simulink model "TLC_Network"  (R2022b)
settings: Solver=VariableStepAuto  StartTime=0.0  StopTime=2  RelTol=1e-3
(part 1 of 2)
settings Model: Creator=Stefano  LastModifiedBy=stefanopanzieri
settings SolverCC: AlgebraicLoopSolver=TrustRegion
settings DebuggingCC: UnconnectedInputMsg=warning  UnconnectedOutputMsg=warning  UnconnectedLineMsg=warning  SFMachineParentedDataDiag=warning
settings ModelReferenceCC: EnableRefExpFcnMdlSchedulingChecks=on
settings SFSimCC: CustomCodeUndefinedFunction=UseInterfaceOnly
settings RTWCC: DLArmComputeVersion=19.05

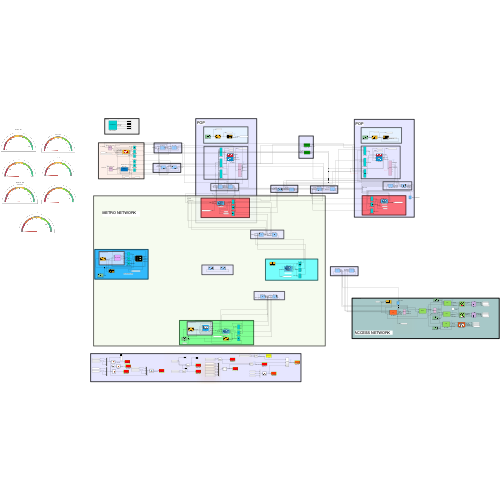
[thumbnail: Simulink's stored preview of the top-level diagram]
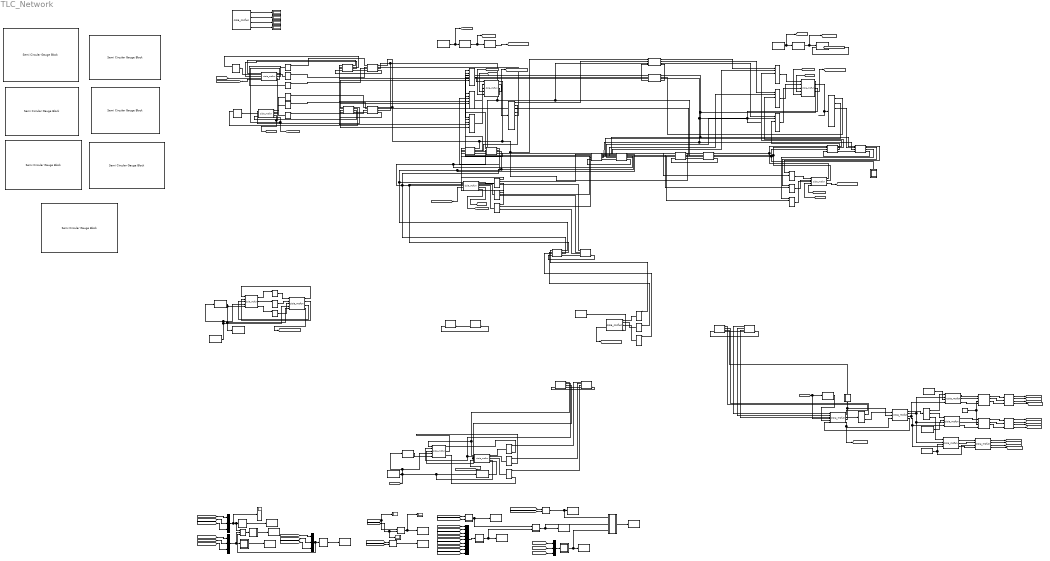
== system TLC_Network ==
  note: POP
  note: ACCESS NETWORK
  note: METRO NETWORK
  note: Web App Firewalls
  note: Core Router/Provider Edge
  note: Distribution Router
  note: Access Router
  note: Border Router
  note: Firewall, IPS/IDS, Malware Detection&Protection
  note: Border Router
  note: Core Network Room
  note: Core Network Room
  note: ACCESS NETWORK
  note: POP
  note: MASTER
  5G_CU_DU_Server_1 (160) : M-S-Function  FunctionName=cisia_msfun  Parameters=Parameter1, Parameter2, Parameter3, resources, Parameter10, codeupdate, step_received, step_computed, dynamic_computed, step_sended, id_entity, id_project, id_type, name_type, color  mask(S-function:msfcn_unit_delay){Parameter1='5G_CU_DU_Server_1', Parameter2=1, Parameter3='ORO', resources=, Parameter10=off, codeupdate=off, step_received=|, step_computed=, dynamic_computed=, step_sended=|, id_entity=160, id_project=6, id_type=40, name_type=App_Server, color=#00AAFF}
      mask step_received=|
      | Connection=max(Connection_init,TLC_CONN);
      | TLC_services=max(TLC_services_init,TLC_SERVICE);
      | TLC_services=mod(TLC_services,10);
      | TLC_revoke=floor(TLC_SERVICE/10);
      |
      | Mechanical_Fault=max([Mechanical_Fault Mechanical_Fault_init]);
      |
      | %if strcmp(name_entity,"BlockChainServer") && (cisia.major_time>=2)
      |  % Dos_attack=1;
      |  %TLC_revoke(9)=1;
      |  %TLC_services(9)=0;
      | %end
      |
      |
      | Cyber_Fault=max(CYBER_FAULT, transpose([Dos_attack   MITM_attack Virus_Attack Port_Scan_Attack  BGP_hijacking BotNet_Attack Data_Corruption SW_Change Config_Change Port_Saturation]));
      |
      | Service_Fault=max(abs(Consumed_Services.*TLC_services-Consumed_Services));
      | Redundancy_Fault=max(abs(Consumed_Services.*TLC_CONN-Consumed_Services));
      |
      | Conn_Fault=max([Dos_attack  Mechanical_Fault  1-POWER 1-ROOM_QoS] );
      |
      |
      | Operative_Level=(1-Conn_Fault)*(1-0.5*max(Cyber_Fault))*(1-Service_Fault)*max(max(TLC_CONN),0.5);
      mask step_sended=|
      | TLC_CONN=Connection*(1-Conn_Fault);
      | TLC_SERVICE=TLC_services*(1-Conn_Fault)*(1-Service_Fault)*(1-syslog_adm_login)+10*TLC_revoke;
      | CYBER_FAULT=Cyber_Fault*(1-Conn_Fault);
      mask prompts: Parameter1 "entity name"; Parameter2 "sampling time"; Parameter3 "project"; resources "input resources and state variables"; Parameter10 "Bring state variables to output"; codeupdate "update code from mask"
      mask help: This is a level-2 MATLAB file S-function which demonstrates CISIA entity
      mask DialogControl Container1 Prompt: All parameters
      mask Display: image('Icons/App_Server.png')
  5G_Core_1 (198) : M-S-Function  FunctionName=cisia_msfun  Parameters=Parameter1, Parameter2, Parameter3, resources, Parameter10, codeupdate, step_received, step_computed, dynamic_computed, step_sended, id_entity, id_project, id_type, name_type, color  mask(S-function:msfcn_unit_delay){Parameter1='5G_Core_1', Parameter2=1, Parameter3='ORO', resources=, Parameter10=off, codeupdate=off, step_received=|, step_computed=, dynamic_computed=, step_sended=|, id_entity=198, id_project=6, id_type=38, name_type=5G_Core, color=#E7A6FF}
      mask step_received=|
      | Connection=max(Connection_init,TLC_CONN);
      | TLC_services=max(TLC_services_init,TLC_SERVICE);
      | TLC_services=mod(TLC_services,10);
      | TLC_revoke=floor(TLC_SERVICE/10);
      | Mechanical_Fault=max([Mechanical_Fault Mechanical_Fault_init]);
      |
      | Cyber_Fault=max(CYBER_FAULT, transpose([Dos_attack   MITM_attack Virus_Attack Port_Scan_Attack  BGP_hijacking BotNet_Attack Data_Corruption SW_Change Config_Change Port_Saturation]));
      |
      |
      |
      | %if (cisia.major_time)>=2
      |    %Dos_attack=1;
      |    %TLC_services(5)=0;
      |   %TLC_revoke(5)=1;
      | %end
      |
      |
      | Conn_Fault=max([Dos_attack  Mechanical_Fault  1-POWER 1-ROOM_QoS] );
      |
      | Service_Fault=max(abs(Consumed_Services.*TLC_services-Consumed_Services));
      | Redundancy_Fault=max(abs(Consumed_Services.*TLC_CONN-Consumed_Services));
      |
      | Operative_Level=(1-Conn_Fault)*(1-0.5*max(Cyber_Fault))*(1-Service_Fault);
      mask step_sended=|
      | TLC_CONN=Connection*(1-Conn_Fault);
      | TLC_SERVICE=TLC_services*(1-Conn_Fault)*(1-Service_Fault)*(1 -syslog_adm_login)+10*TLC_revoke;
      | %TLC_SERVICE=TLC_services
      | CYBER_FAULT=Cyber_Fault*(1-Conn_Fault);
      mask prompts: Parameter1 "entity name"; Parameter2 "sampling time"; Parameter3 "project"; resources "input resources and state variables"; Parameter10 "Bring state variables to output"; codeupdate "update code from mask"
      mask help: This is a level-2 MATLAB file S-function which demonstrates CISIA entity
      mask DialogControl Container1 Prompt: All parameters
      mask Display: disp('RFI_Sist_Informativo_1')
  ANTENNA_1 (56) : M-S-Function  FunctionName=cisia_msfun  Parameters=Parameter1, Parameter2, Parameter3, resources, Parameter10, codeupdate, step_received, step_computed, dynamic_computed, step_sended, id_entity, id_project, id_type, name_type, color  mask(S-function:msfcn_unit_delay){Parameter1='ANTENNA_1', Parameter2=1, Parameter3='ORO', resources=, Parameter10=off, codeupdate=off, step_received=|, step_computed=, dynamic_computed=, step_sended=|, id_entity=56, id_project=6, id_type=13, name_type=RU-DU_ANTENNA, color=#90DB5A}
      mask step_received=|
      | Connection=max(Connection_init,NGPON_CONN);
      | TLC_services=max(TLC_services_init,TLC_SERVICE);
      | TLC_services=mod(TLC_services,10);
      | TLC_revoke=floor(TLC_SERVICE/10);
      |
      | Cyber_Fault=max(CYBER_FAULT, transpose([Dos_attack   MITM_attack Virus_Attack Port_Scan_Attack  BGP_hijacking BotNet_Attack Data_Corruption SW_Change Config_Change Port_Saturation]));
      |
      | % Vale 1 in presenza di fault
      | Conn_Fault=max([Dos_attack  Mechanical_Fault  1-POWER] );
      |
      | Service_Fault=max(abs(Consumed_Services.*TLC_services-Consumed_Services));
      | Redundancy_Fault=max(abs(Consumed_Services.*NGPON_CONN-Consumed_Services));
      |
      |
      | Operative_Level=(1-Conn_Fault)*max(max(NGPON_CONN),0.5)*((2*(1-Service_Fault)+(1-Redundancy_Fault))/3);
      |
      | % Il servizio utilizzato
      | My_Service=max([(1-Service_Fault) (1-Redundancy_Fault)/2]);
      mask step_sended=|
      | R_CONN=Connection*(1-Conn_Fault);
      | TLC_SERVICE=TLC_services*(1-Conn_Fault)+10*TLC_revoke;
      |
      | Cyber_Transmitted=min(Cyber_Fault, transpose([0 0 1 0 1 1 0 0 0 1]));
      | CYBER_FAULT=Cyber_Transmitted*(1-Conn_Fault);
      |
      |
      | RF_QoS=My_Service;
      mask prompts: Parameter1 "entity name"; Parameter2 "sampling time"; Parameter3 "project"; resources "input resources and state variables"; Parameter10 "Bring state variables to output"; codeupdate "update code from mask"
      mask help: This is a level-2 MATLAB file S-function which demonstrates CISIA entity
      mask DialogControl Container1 Prompt: All parameters
      mask Display: image('Icons/RU-DU_ANTENNA.png')
  ANTENNA_2 (60) : M-S-Function  FunctionName=cisia_msfun  Parameters=Parameter1, Parameter2, Parameter3, resources, Parameter10, codeupdate, step_received, step_computed, dynamic_computed, step_sended, id_entity, id_project, id_type, name_type, color  mask(S-function:msfcn_unit_delay){Parameter1='ANTENNA_2', Parameter2=1, Parameter3='ORO', resources=, Parameter10=off, codeupdate=off, step_received=|, step_computed=, dynamic_computed=, step_sended=|, id_entity=60, id_project=6, id_type=13, name_type=RU-DU_ANTENNA, color=#90DB5A}
      mask step_received=|
      | Connection=max(Connection_init,NGPON_CONN);
      | TLC_services=max(TLC_services_init,TLC_SERVICE);
      | TLC_services=mod(TLC_services,10);
      | TLC_revoke=floor(TLC_SERVICE/10);
      |
      | Cyber_Fault=max(CYBER_FAULT, transpose([Dos_attack   MITM_attack Virus_Attack Port_Scan_Attack  BGP_hijacking BotNet_Attack Data_Corruption SW_Change Config_Change Port_Saturation]));
      |
      | % Vale 1 in presenza di fault
      | Conn_Fault=max([Dos_attack  Mechanical_Fault  1-POWER] );
      |
      | Service_Fault=max(abs(Consumed_Services.*TLC_services-Consumed_Services));
      | Redundancy_Fault=max(abs(Consumed_Services.*NGPON_CONN-Consumed_Services));
      |
      |
      | Operative_Level=(1-Conn_Fault)*max(max(NGPON_CONN),0.5)*((2*(1-Service_Fault)+(1-Redundancy_Fault))/3);
      |
      | % Il servizio utilizzato
      | My_Service=max([(1-Service_Fault) (1-Redundancy_Fault)/2]);
      mask step_sended=|
      | R_CONN=Connection*(1-Conn_Fault);
      | TLC_SERVICE=TLC_services*(1-Conn_Fault)+10*TLC_revoke;
      |
      | Cyber_Transmitted=min(Cyber_Fault, transpose([0 0 1 0 1 1 0 0 0 1]));
      | CYBER_FAULT=Cyber_Transmitted*(1-Conn_Fault);
      |
      |
      | RF_QoS=My_Service;
      mask prompts: Parameter1 "entity name"; Parameter2 "sampling time"; Parameter3 "project"; resources "input resources and state variables"; Parameter10 "Bring state variables to output"; codeupdate "update code from mask"
      mask help: This is a level-2 MATLAB file S-function which demonstrates CISIA entity
      mask DialogControl Container1 Prompt: All parameters
      mask Display: image('Icons/RU-DU_ANTENNA.png')
  ASR9006_1 (9) : M-S-Function  FunctionName=cisia_msfun  Parameters=Parameter1, Parameter2, Parameter3, resources, Parameter10, codeupdate, step_received, step_computed, dynamic_computed, step_sended, id_entity, id_project, id_type, name_type, color  mask(S-function:msfcn_unit_delay){Parameter1='ASR9006_1', Parameter2=1, Parameter3='ORO', resources=, Parameter10=off, codeupdate=off, step_received=|, step_computed=, dynamic_computed=, step_sended=|, id_entity=9, id_project=6, id_type=3, name_type=CISCO_router, color=#4DBEEE}
      mask step_received=|
      | Connection=max(Connection_init,TLC_CONN);
      | TLC_services=max(TLC_services_init,TLC_SERVICE);
      | TLC_services=mod(TLC_services,10);
      | TLC_revoke=floor(TLC_SERVICE/10);
      |
      | Cyber_Fault=max(CYBER_FAULT, transpose([Dos_attack   MITM_attack Virus_Attack Port_Scan_Attack  BGP_hijacking BotNet_Attack Data_Corruption SW_Change Config_Change Port_Saturation]));
      |
      |
      | Conn_Fault=max([Dos_attack BGP_hijacking Route_Poisoning Interface_Down Mechanical_Fault  1-POWER 1-ROOM_QoS Earthquake_Fault] );
      |
      | Room_Fault=1-ROOM_QoS;
      |
      | Operative_Level=(1-Room_Fault)*(1-Conn_Fault)*max(max(TLC_services),0.5)*(1-0.5*max(Cyber_Fault));
      mask step_sended=|
      | TLC_CONN=Connection*(1-Conn_Fault);
      | TLC_SERVICE=TLC_services*(1-Room_Fault)*(1-Conn_Fault)*(1-syslog_adm_login)+10*TLC_revoke;
      |
      |
      | Cyber_Transmitted=min(Cyber_Fault, transpose([0 0 1 0 1 1 0 0 0 1]));
      |
      | CYBER_FAULT=Cyber_Transmitted*(1-Conn_Fault);
      |
      | ROUTING_QoS=Operative_Level;
      mask prompts: Parameter1 "entity name"; Parameter2 "sampling time"; Parameter3 "project"; resources "input resources and state variables"; Parameter10 "Bring state variables to output"; codeupdate "update code from mask"
      mask help: This is a level-2 MATLAB file S-function which demonstrates CISIA entity
      mask DialogControl Container1 Prompt: All parameters
      mask Display: image('Icons/CISCO_router.png')
  ASR9006_2 (10) : M-S-Function  FunctionName=cisia_msfun  Parameters=Parameter1, Parameter2, Parameter3, resources, Parameter10, codeupdate, step_received, step_computed, dynamic_computed, step_sended, id_entity, id_project, id_type, name_type, color  mask(S-function:msfcn_unit_delay){Parameter1='ASR9006_2', Parameter2=1, Parameter3='ORO', resources=, Parameter10=off, codeupdate=off, step_received=|, step_computed=, dynamic_computed=, step_sended=|, id_entity=10, id_project=6, id_type=3, name_type=CISCO_router, color=#4DBEEE}
      mask step_received=|
      | Connection=max(Connection_init,TLC_CONN);
      | TLC_services=max(TLC_services_init,TLC_SERVICE);
      | TLC_services=mod(TLC_services,10);
      | TLC_revoke=floor(TLC_SERVICE/10);
      |
      | Cyber_Fault=max(CYBER_FAULT, transpose([Dos_attack   MITM_attack Virus_Attack Port_Scan_Attack  BGP_hijacking BotNet_Attack Data_Corruption SW_Change Config_Change Port_Saturation]));
      |
      |
      | Conn_Fault=max([Dos_attack BGP_hijacking Route_Poisoning Interface_Down Mechanical_Fault  1-POWER 1-ROOM_QoS Earthquake_Fault] );
      |
      | Room_Fault=1-ROOM_QoS;
      |
      | Operative_Level=(1-Room_Fault)*(1-Conn_Fault)*max(max(TLC_services),0.5)*(1-0.5*max(Cyber_Fault));
      mask step_sended=|
      | TLC_CONN=Connection*(1-Conn_Fault);
      | TLC_SERVICE=TLC_services*(1-Room_Fault)*(1-Conn_Fault)*(1-syslog_adm_login)+10*TLC_revoke;
      |
      |
      | Cyber_Transmitted=min(Cyber_Fault, transpose([0 0 1 0 1 1 0 0 0 1]));
      |
      | CYBER_FAULT=Cyber_Transmitted*(1-Conn_Fault);
      |
      | ROUTING_QoS=Operative_Level;
      mask prompts: Parameter1 "entity name"; Parameter2 "sampling time"; Parameter3 "project"; resources "input resources and state variables"; Parameter10 "Bring state variables to output"; codeupdate "update code from mask"
      mask help: This is a level-2 MATLAB file S-function which demonstrates CISIA entity
      mask DialogControl Container1 Prompt: All parameters
      mask Display: image('Icons/CISCO_router.png')
  ASR903_1 (5) : M-S-Function  FunctionName=cisia_msfun  Parameters=Parameter1, Parameter2, Parameter3, resources, Parameter10, codeupdate, step_received, step_computed, dynamic_computed, step_sended, id_entity, id_project, id_type, name_type, color  mask(S-function:msfcn_unit_delay){Parameter1='ASR903_1', Parameter2=1, Parameter3='ORO', resources=, Parameter10=off, codeupdate=off, step_received=|, step_computed=, dynamic_computed=, step_sended=|, id_entity=5, id_project=6, id_type=3, name_type=CISCO_router, color=#4DBEEE}
      mask step_received=|
      | Connection=max(Connection_init,TLC_CONN);
      | TLC_services=max(TLC_services_init,TLC_SERVICE);
      | TLC_services=mod(TLC_services,10);
      | TLC_revoke=floor(TLC_SERVICE/10);
      |
      | Cyber_Fault=max(CYBER_FAULT, transpose([Dos_attack   MITM_attack Virus_Attack Port_Scan_Attack  BGP_hijacking BotNet_Attack Data_Corruption SW_Change Config_Change Port_Saturation]));
      |
      |
      | Conn_Fault=max([Dos_attack BGP_hijacking Route_Poisoning Interface_Down Mechanical_Fault  1-POWER 1-ROOM_QoS Earthquake_Fault] );
      |
      | Room_Fault=1-ROOM_QoS;
      |
      | Operative_Level=(1-Room_Fault)*(1-Conn_Fault)*max(max(TLC_services),0.5)*(1-0.5*max(Cyber_Fault));
      mask step_sended=|
      | TLC_CONN=Connection*(1-Conn_Fault);
      | TLC_SERVICE=TLC_services*(1-Room_Fault)*(1-Conn_Fault)*(1-syslog_adm_login)+10*TLC_revoke;
      |
      |
      | Cyber_Transmitted=min(Cyber_Fault, transpose([0 0 1 0 1 1 0 0 0 1]));
      |
      | CYBER_FAULT=Cyber_Transmitted*(1-Conn_Fault);
      |
      | ROUTING_QoS=Operative_Level;
      mask prompts: Parameter1 "entity name"; Parameter2 "sampling time"; Parameter3 "project"; resources "input resources and state variables"; Parameter10 "Bring state variables to output"; codeupdate "update code from mask"
      mask help: This is a level-2 MATLAB file S-function which demonstrates CISIA entity
      mask DialogControl Container1 Prompt: All parameters
      mask Display: image('Icons/CISCO_router.png')
  ASR920_1 (7) : M-S-Function  FunctionName=cisia_msfun  Parameters=Parameter1, Parameter2, Parameter3, resources, Parameter10, codeupdate, step_received, step_computed, dynamic_computed, step_sended, id_entity, id_project, id_type, name_type, color  mask(S-function:msfcn_unit_delay){Parameter1='ASR920_1', Parameter2=1, Parameter3='ORO', resources=, Parameter10=off, codeupdate=off, step_received=|, step_computed=, dynamic_computed=, step_sended=|, id_entity=7, id_project=6, id_type=3, name_type=CISCO_router, color=#4DBEEE}
      mask step_received=|
      | Connection=max(Connection_init,TLC_CONN);
      | TLC_services=max(TLC_services_init,TLC_SERVICE);
      | TLC_services=mod(TLC_services,10);
      | TLC_revoke=floor(TLC_SERVICE/10);
      |
      | Cyber_Fault=max(CYBER_FAULT, transpose([Dos_attack   MITM_attack Virus_Attack Port_Scan_Attack  BGP_hijacking BotNet_Attack Data_Corruption SW_Change Config_Change Port_Saturation]));
      |
      |
      | Conn_Fault=max([Dos_attack BGP_hijacking Route_Poisoning Interface_Down Mechanical_Fault  1-POWER 1-ROOM_QoS Earthquake_Fault] );
      |
      | Room_Fault=1-ROOM_QoS;
      |
      | Operative_Level=(1-Room_Fault)*(1-Conn_Fault)*max(max(TLC_services),0.5)*(1-0.5*max(Cyber_Fault));
      mask step_sended=|
      | TLC_CONN=Connection*(1-Conn_Fault);
      | TLC_SERVICE=TLC_services*(1-Room_Fault)*(1-Conn_Fault)*(1-syslog_adm_login)+10*TLC_revoke;
      |
      |
      | Cyber_Transmitted=min(Cyber_Fault, transpose([0 0 1 0 1 1 0 0 0 1]));
      |
      | CYBER_FAULT=Cyber_Transmitted*(1-Conn_Fault);
      |
      | ROUTING_QoS=Operative_Level;
      mask prompts: Parameter1 "entity name"; Parameter2 "sampling time"; Parameter3 "project"; resources "input resources and state variables"; Parameter10 "Bring state variables to output"; codeupdate "update code from mask"
      mask help: This is a level-2 MATLAB file S-function which demonstrates CISIA entity
      mask DialogControl Container1 Prompt: All parameters
      mask Display: image('Icons/CISCO_router.png')
  Alcatel_1 (26) : M-S-Function  FunctionName=cisia_msfun  Parameters=Parameter1, Parameter2, Parameter3, resources, Parameter10, codeupdate, step_received, step_computed, dynamic_computed, step_sended, id_entity, id_project, id_type, name_type, color  mask(S-function:msfcn_unit_delay){Parameter1='Alcatel_1', Parameter2=1, Parameter3='ORO', resources=, Parameter10=off, codeupdate=off, step_received=|, step_computed=, dynamic_computed=, step_sended=|, id_entity=26, id_project=6, id_type=5, name_type=Alcatel7750, color=#ACBD7E}
      mask step_received=|
      | Connection=max(Connection_init,TLC_CONN);
      | TLC_services=max(TLC_services_init,TLC_SERVICE);
      | TLC_services=mod(TLC_services,10);
      | TLC_revoke=floor(TLC_SERVICE/10);
      |
      | Cyber_Fault=max(CYBER_FAULT, transpose([Dos_attack   MITM_attack Virus_Attack Port_Scan_Attack  BGP_hijacking BotNet_Attack Data_Corruption SW_Change Config_Change Port_Saturation]));
      |
      | Conn_Fault=max([Dos_attack  Mechanical_Fault  1-POWER 1-ROOM_QoS] );
      |
      |
      | Operative_Level=(1-Conn_Fault)*(1-0.5*max(Cyber_Fault))*max(max(TLC_services),0.5);
      mask step_sended=|
      | TLC_CONN=Connection*(1-Conn_Fault);
      | TLC_SERVICE=TLC_services*(1-Conn_Fault)+TLC_revoke*10;
      | CYBER_FAULT=Cyber_Fault*(1-Conn_Fault);
      |
      | ROUTING_QoS=Operative_Level;
      mask prompts: Parameter1 "entity name"; Parameter2 "sampling time"; Parameter3 "project"; resources "input resources and state variables"; Parameter10 "Bring state variables to output"; codeupdate "update code from mask"
      mask help: This is a level-2 MATLAB file S-function which demonstrates CISIA entity
      mask DialogControl Container1 Prompt: All parameters
      mask Display: image('Icons/Alcatel7750.png')
  BIGP_2 (35) : M-S-Function  FunctionName=cisia_msfun  Parameters=Parameter1, Parameter2, Parameter3, resources, Parameter10, codeupdate, step_received, step_computed, dynamic_computed, step_sended, id_entity, id_project, id_type, name_type, color  mask(S-function:msfcn_unit_delay){Parameter1='BIGP_2', Parameter2=1, Parameter3='ORO', resources=, Parameter10=off, codeupdate=off, step_received=|, step_computed=, dynamic_computed=, step_sended=|, id_entity=35, id_project=6, id_type=7, name_type=F5BIGP, color=#0072BD}
      mask step_received=|
      | Connection=max(Connection_init,TLC_CONN);
      | TLC_services=max(TLC_services_init,TLC_SERVICE);
      | TLC_services=mod(TLC_services,10);
      | TLC_revoke=floor(TLC_SERVICE/10);
      |
      | Cyber_Fault=max(CYBER_FAULT, transpose([Dos_attack   MITM_attack Virus_Attack Port_Scan_Attack  BGP_hijacking BotNet_Attack Data_Corruption SW_Change Config_Change Port_Saturation]));
      |
      | Conn_Fault=max([Dos_attack  Mechanical_Fault  1-POWER 1-ROOM_QoS] );
      |
      | Service_Fault=max(abs(Consumed_Services.*TLC_services-Consumed_Services));
      | Redundancy_Fault=max(abs(Consumed_Services.*TLC_CONN-Consumed_Services));
      |
      | %Operative_Level=(1-Conn_Fault)*((2*(1-Service_Fault)+(1-Redundancy_Fault))/3);
      | Operative_Level=(1-Conn_Fault)*(1-0.5*max(Cyber_Fault))*(1-Service_Fault)*max(max(TLC_CONN),0.5);
      mask step_sended=|
      | TLC_CONN=Connection*(1-Conn_Fault);
      | TLC_SERVICE=TLC_services*(1-Conn_Fault)*(1-Service_Fault)+10*TLC_revoke;
      |
      | Cyber_Transmitted=min(Cyber_Fault, transpose([0 0 1 0 1 1 0 0 0 1]));
      |
      | CYBER_FAULT=Cyber_Transmitted*(1-Conn_Fault);
      mask prompts: Parameter1 "entity name"; Parameter2 "sampling time"; Parameter3 "project"; resources "input resources and state variables"; Parameter10 "Bring state variables to output"; codeupdate "update code from mask"
      mask help: This is a level-2 MATLAB file S-function which demonstrates CISIA entity
      mask DialogControl Container1 Prompt: All parameters
      mask Display: disp('F5BIGP')
  BLM_1500 (91) : M-S-Function  FunctionName=cisia_msfun  Parameters=Parameter1, Parameter2, Parameter3, resources, Parameter10, codeupdate, step_received, step_computed, dynamic_computed, step_sended, id_entity, id_project, id_type, name_type, color  mask(S-function:msfcn_unit_delay){Parameter1='BLM_1500', Parameter2=1, Parameter3='ORO', resources=, Parameter10=off, codeupdate=off, step_received=|, step_computed=, dynamic_computed=, step_sended=|, id_entity=91, id_project=6, id_type=4, name_type=OLT, color=#FF6929}
      mask step_received=|
      | Connection=max(Connection_init,TLC_CONN);
      | TLC_services=max(TLC_services_init,TLC_SERVICE);
      | TLC_services=mod(TLC_services,10);
      | TLC_revoke=floor(TLC_SERVICE/10);
      |
      | Cyber_Fault=max(CYBER_FAULT, transpose([Dos_attack   MITM_attack Virus_Attack Port_Scan_Attack  BGP_hijacking BotNet_Attack Data_Corruption SW_Change Config_Change Port_Saturation]));
      |
      |
      | % Vale 1 in presenza di fault
      | Conn_Fault=max([Dos_attack  Mechanical_Fault  1-POWER 1-ROOM_QoS] );
      |
      |
      | Service_Fault=max(abs(Consumed_Services.*TLC_services-Consumed_Services));
      |
      |
      | Redundancy_Fault=max(abs(Consumed_Services.*TLC_CONN-Consumed_Services));
      |
      | Operative_Level=(1-Conn_Fault)*(1-0.5*max(Cyber_Fault))*(1-Service_Fault)*max(max(TLC_CONN),0.5);
      |
      |
      | %Operative_Level=(1-Conn_Fault)*max(max(TLC_CONN),0.5)*((2*(1-Service_Fault)+(1-Redundancy_Fault))/3);
      | %My_Service=max([(1-Service_Fault) (1-Redundancy_Fault)/2]);
      | %Operative_Level=(1-Conn_Fault)*My_Service;
      mask step_sended=|
      | TLC_CONN=Connection*(1-Conn_Fault);
      | TLC_SERVICE=TLC_services*(1-Conn_Fault)+10*TLC_revoke;
      |
      | Cyber_Transmitted=min(Cyber_Fault, transpose([0 0 1 0 1 1 0 0 0 1]));
      | CYBER_FAULT=Cyber_Transmitted*(1-Conn_Fault);
      |
      | NGPON_CONN=TLC_CONN;
      mask prompts: Parameter1 "entity name"; Parameter2 "sampling time"; Parameter3 "project"; resources "input resources and state variables"; Parameter10 "Bring state variables to output"; codeupdate "update code from mask"
      mask help: This is a level-2 MATLAB file S-function which demonstrates CISIA entity
      mask DialogControl Container1 Prompt: All parameters
      mask Display: disp('OLT')
  Building_1 (53) : M-S-Function  FunctionName=cisia_msfun  Parameters=Parameter1, Parameter2, Parameter3, resources, Parameter10, codeupdate, step_received, step_computed, dynamic_computed, step_sended, id_entity, id_project, id_type, name_type, color  mask(S-function:msfcn_unit_delay){Parameter1='Building_1', Parameter2=1, Parameter3='ORO', resources=, Parameter10=off, codeupdate=off, step_received=|, step_computed=, dynamic_computed=, step_sended=|, id_entity=53, id_project=6, id_type=10, name_type=Building, color=#AB7A07}
      mask step_received=|
      | Physical_Fault=max([Unauthorized_Access Perimeter_Security_Fault Security_Camera_Fault Earthquake_Fault]);
      |
      | Conn_Fault=max([Power_Fault 1-ROOM_QoS]);
      |
      | Operative_Level=min([ (1-Physical_Fault) (1-Conn_Fault) (1-Perimeter_Security_Fault) (1-Earthquake_Fault) ]);
      mask step_sended=|
      | BUILDING_QoS=Operative_Level;
      |
      | %Cyber_Fault=0.3*ones(size(Cyber_Fault));
      |
      | CYBER_FAULT=Perimeter_Security_Fault*Cyber_Fault;
      mask prompts: Parameter1 "entity name"; Parameter2 "sampling time"; Parameter3 "project"; resources "input resources and state variables"; Parameter10 "Bring state variables to output"; codeupdate "update code from mask"
      mask help: This is a level-2 MATLAB file S-function which demonstrates CISIA entity
      mask DialogControl Container1 Prompt: All parameters
      mask Display: image('Icons/Building.png')
  Building_2 (201) : M-S-Function  FunctionName=cisia_msfun  Parameters=Parameter1, Parameter2, Parameter3, resources, Parameter10, codeupdate, step_received, step_computed, dynamic_computed, step_sended, id_entity, id_project, id_type, name_type, color  mask(S-function:msfcn_unit_delay){Parameter1='Building_2', Parameter2=1, Parameter3='ORO', resources=, Parameter10=off, codeupdate=off, step_received=|, step_computed=, dynamic_computed=, step_sended=|, id_entity=201, id_project=6, id_type=10, name_type=Building, color=#AB7A07}
      mask step_received=|
      | Physical_Fault=max([Unauthorized_Access Perimeter_Security_Fault Security_Camera_Fault Earthquake_Fault]);
      |
      | Conn_Fault=max([Power_Fault 1-ROOM_QoS]);
      |
      | Operative_Level=min([ (1-Physical_Fault) (1-Conn_Fault) (1-Perimeter_Security_Fault) (1-Earthquake_Fault) ]);
      mask step_sended=|
      | BUILDING_QoS=Operative_Level;
      |
      | %Cyber_Fault=0.3*ones(size(Cyber_Fault));
      |
      | CYBER_FAULT=Perimeter_Security_Fault*Cyber_Fault;
      mask prompts: Parameter1 "entity name"; Parameter2 "sampling time"; Parameter3 "project"; resources "input resources and state variables"; Parameter10 "Bring state variables to output"; codeupdate "update code from mask"
      mask help: This is a level-2 MATLAB file S-function which demonstrates CISIA entity
      mask DialogControl Container1 Prompt: All parameters
      mask Display: image('Icons/Building.png')
  Building_3 (215) : M-S-Function  FunctionName=cisia_msfun  Parameters=Parameter1, Parameter2, Parameter3, resources, Parameter10, codeupdate, step_received, step_computed, dynamic_computed, step_sended, id_entity, id_project, id_type, name_type, color  mask(S-function:msfcn_unit_delay){Parameter1='Building_3', Parameter2=1, Parameter3='ORO', resources=, Parameter10=off, codeupdate=off, step_received=|, step_computed=, dynamic_computed=, step_sended=|, id_entity=215, id_project=6, id_type=10, name_type=Building, color=#AB7A07}
      mask step_received=|
      | Physical_Fault=max([Unauthorized_Access Perimeter_Security_Fault Security_Camera_Fault Earthquake_Fault]);
      |
      | Conn_Fault=max([Power_Fault 1-ROOM_QoS]);
      |
      | Operative_Level=min([ (1-Physical_Fault) (1-Conn_Fault) (1-Perimeter_Security_Fault) (1-Earthquake_Fault) ]);
      mask step_sended=|
      | BUILDING_QoS=Operative_Level;
      |
      | %Cyber_Fault=0.3*ones(size(Cyber_Fault));
      |
      | CYBER_FAULT=Perimeter_Security_Fault*Cyber_Fault;
      mask prompts: Parameter1 "entity name"; Parameter2 "sampling time"; Parameter3 "project"; resources "input resources and state variables"; Parameter10 "Bring state variables to output"; codeupdate "update code from mask"
      mask help: This is a level-2 MATLAB file S-function which demonstrates CISIA entity
      mask DialogControl Container1 Prompt: All parameters
      mask Display: image('Icons/Building.png')
  CISIA_MASTER (0) : M-S-Function  FunctionName=cisia_msfun  Parameters=Parameter1, Parameter2, Parameter3, resources, Parameter4, Parameter5, Parameter6, Parameter7, Parameter8, Parameter9,Parameter11  mask(S-function:msfcn_unit_delay){Parameter1='CISIA_MASTER', Parameter2=1, Parameter3='Iside', resources=off, Parameter4=on, Parameter5=off, Parameter6=off, Parameter7=off, Parameter8=0.001, Parameter9=off, Parameter11=on}
      mask prompts: Parameter1 "entity name"; Parameter2 "sampling time"; Parameter3 "project"; resources "Save status at each major hit"; Parameter4 "Show Operative Levels with colors"; Parameter5 "Load Entities from file"; Parameter6 "Load Start from Mask"; Parameter7 "Real Time"; Parameter8 "Real Time Hit (sec)"; Parameter9 "Skip saving"; Parameter11 "Show unconnected"
      mask help: This is a level-2 MATLAB file S-function which demonstrates CISIA entity
      mask Display: disp('MASTER BLOCK')
  CYBER_fault1 : MinMax  Function=max  Inputs=6
  CYBER_fault12 : MinMax  Function=max  Inputs=2
  CYBER_fault13 : MinMax  Function=max  Inputs=2
  CYBER_fault2 : MinMax  Function=max  Inputs=6
  CYBER_fault{3..5,8} (4 alike) : MinMax  Function=max  Inputs=4
  CYBER_fault9 : MinMax  Function=max  Inputs=2
  Constant : Constant
  Display{1..4,9,15..17} (8 alike) : Display
  FG1500_2 (33) : M-S-Function  FunctionName=cisia_msfun  Parameters=Parameter1, Parameter2, Parameter3, resources, Parameter10, codeupdate, step_received, step_computed, dynamic_computed, step_sended, id_entity, id_project, id_type, name_type, color  mask(S-function:msfcn_unit_delay){Parameter1='FG1500_2', Parameter2=1, Parameter3='ORO', resources=, Parameter10=off, codeupdate=off, step_received=|, step_computed=, dynamic_computed=, step_sended=|, id_entity=33, id_project=6, id_type=6, name_type=FortiGate1500D, color=#EDB120}
      mask step_received=|
      | Connection=max(Connection_init,TLC_CONN);
      | TLC_services=max(TLC_services_init,TLC_SERVICE);
      | TLC_services=mod(TLC_services,10);
      | TLC_revoke=floor(TLC_SERVICE/10);
      |
      | Cyber_Fault=max(CYBER_FAULT, transpose([Dos_attack   MITM_attack Virus_Attack Port_Scan_Attack  BGP_hijacking BotNet_Attack Data_Corruption SW_Change Config_Change Port_Saturation]));
      |
      | Conn_Fault=max([Dos_attack  Mechanical_Fault  1-POWER 1-ROOM_QoS  0.5*max(Cyber_Fault)] );
      |
      | Service_Fault=max(abs(Consumed_Services.*TLC_services-Consumed_Services));
      | Redundancy_Fault=max(abs(Consumed_Services.*TLC_CONN-Consumed_Services));
      |
      | %Operative_Level=(1-Conn_Fault)*((2*(1-Service_Fault)+(1-Redundancy_Fault))/3);
      | Operative_Level=(1-Conn_Fault)*(1-0.5*max(Cyber_Fault))*(1-Service_Fault)*max(max(TLC_CONN),0.5);
      mask step_sended=|
      | TLC_CONN=Connection*(1-Conn_Fault);
      | TLC_SERVICE=TLC_services*(1-Conn_Fault)*(1-Service_Fault)+10*TLC_revoke;
      |
      | Cyber_Transmitted=min(Cyber_Fault, transpose([0 0 1 0 1 1 0 0 0 1]));
      | CYBER_FAULT=Cyber_Transmitted*(1-Conn_Fault);
      |
      | FIREWALL_QoS=(1-Service_Fault)*(1-Conn_Fault);
      | REDUNDANCY_QoS=(1-Redundancy_Fault);
      mask prompts: Parameter1 "entity name"; Parameter2 "sampling time"; Parameter3 "project"; resources "input resources and state variables"; Parameter10 "Bring state variables to output"; codeupdate "update code from mask"
      mask help: This is a level-2 MATLAB file S-function which demonstrates CISIA entity
      mask DialogControl Container1 Prompt: All parameters
      mask Display: image('Icons/FortiGate1500D.png')
  Half Gauge{1..7} (7 alike) : SemiCircularGaugeBlock  ScaleMax=1
  House_1 (145) : M-S-Function  FunctionName=cisia_msfun  Parameters=Parameter1, Parameter2, Parameter3, resources, Parameter10, codeupdate, step_received, step_computed, dynamic_computed, step_sended, id_entity, id_project, id_type, name_type, color  mask(S-function:msfcn_unit_delay){Parameter1='House_1', Parameter2=1, Parameter3='ORO', resources=, Parameter10=off, codeupdate=off, step_received=|, step_computed=, dynamic_computed=, step_sended=|, id_entity=145, id_project=6, id_type=37, name_type=House, color=#D95319}
      mask step_received=|
      | Connection=max(Connection_init,NGPON_CONN);
      | TLC_services=max(TLC_services_init,TLC_SERVICE);
      | TLC_services=mod(TLC_services,10);
      | TLC_revoke=floor(TLC_SERVICE/10);
      |
      | Cyber_Fault=max(CYBER_FAULT, transpose([Dos_attack   MITM_attack Virus_Attack Port_Scan_Attack  BGP_hijacking BotNet_Attack Data_Corruption SW_Change Config_Change Port_Saturation]));
      |
      | % Vale 1 in presenza di fault
      | Conn_Fault=max([Dos_attack  Mechanical_Fault  1-POWER] );
      |
      | Service_Fault=max(abs(Consumed_Services.*TLC_services-Consumed_Services));
      | Redundancy_Fault=max(abs(Consumed_Services.*NGPON_CONN-Consumed_Services));
      |
      | Alt_Serv_Fault=max(abs(Alternative_Services.*NGPON_CONN-Alternative_Services));
      |
      | Alt_Rout_Fault=max(abs(Consumed_Services.*NGPON_CONN-Consumed_Services));
      |
      | Port_Isolation=min(max(transpose([1 1 1 1 1 1 1 1 1 0]), CYBER_FAULT));
      |
      |
      | Operative_Level=(1-Conn_Fault)*max(max(NGPON_CONN),0.5)*(((1-Service_Fault)+(1-Redundancy_Fault)+(1-Port_Isolation))/3);
      |
      | Alt_Port_Isol=(1-Conn_Fault)*max(max(NGPON_CONN),0.5)*(((1-Service_Fault)+(1-Redundancy_Fault))/2);
      |
      |
      | % Il servizio utilizzato
      | My_Service=max([(1-Service_Fault) (1-Redundancy_Fault)/2]);
      mask step_sended=|
      | HOME_QoS=My_Service;
      |
      | ALT_SERVICES=1-Alt_Serv_Fault;
      |
      | ALT_ROUTING=1-Alt_Rout_Fault;
      |
      | ALT_PORT_ISOLATION=Alt_Port_Isol;
      mask prompts: Parameter1 "entity name"; Parameter2 "sampling time"; Parameter3 "project"; resources "input resources and state variables"; Parameter10 "Bring state variables to output"; codeupdate "update code from mask"
      mask help: This is a level-2 MATLAB file S-function which demonstrates CISIA entity
      mask DialogControl Container1 Prompt: All parameters
      mask Display: image('Icons/House.png')
  Mask Port Saturation : Subsystem  mask{Mask_value=[1 1 1 1 1 1 1 1 1 0]}
      mask prompts: Mask_value "Mask value"
  Mask Port Saturation2 : Subsystem  mask{Mask_value=[1 1 1 1 1 1 1 1 1 0]}
      mask prompts: Mask_value "Mask value"
  Max : MinMax  Function=max  Inputs=3
  Mobile_1 (147) : M-S-Function  FunctionName=cisia_msfun  Parameters=Parameter1, Parameter2, Parameter3, resources, Parameter10, codeupdate, step_received, step_computed, dynamic_computed, step_sended, id_entity, id_project, id_type, name_type, color  mask(S-function:msfcn_unit_delay){Parameter1='Mobile_1', Parameter2=1, Parameter3='ORO', resources=, Parameter10=off, codeupdate=off, step_received=|, step_computed=, dynamic_computed=, step_sended=|, id_entity=147, id_project=6, id_type=39, name_type=MobileUnit, color=#C9ABDB}
      mask step_received=|
      | Connection=max(Connection_init,R_CONN);
      | TLC_services=max(TLC_services_init,TLC_SERVICE);
      | TLC_services=mod(TLC_services,10);
      | TLC_revoke=floor(TLC_SERVICE/10);
      |
      | Service_Fault=max(abs(Consumed_Services.*TLC_services-Consumed_Services));
      | Redundancy_Fault=max(abs(Consumed_Services.*R_CONN-Consumed_Services));
      |
      | Alt_Serv_Fault=max(abs(Alternative_Services.*R_CONN-Alternative_Services));
      |
      | Alt_Rout_Fault=max(abs(Consumed_Services.*R_CONN-Consumed_Services));
      |
      | Port_Isolation=min(max(transpose([1 1 1 1 1 1 1 1 1 0]), CYBER_FAULT));
      |
      |
      | Operative_Level=(1-Mechanical_Fault)*max(max(R_CONN), 0.5)*(((1-Service_Fault)+(1-Redundancy_Fault)+(1-Port_Isolation))/3);
      |
      | Alt_Port_Isol=(1-Mechanical_Fault)*max(max(R_CONN), 0.5)*(((1-Service_Fault)+(1-Redundancy_Fault))/2);
      mask step_sended=|
      | MOBILE_QoS=Operative_Level;
      |
      |
      | ALT_SERVICES=1-Alt_Serv_Fault;
      | ALT_ROUTING=1-Alt_Rout_Fault;
      | ALT_PORT_ISOLATION=Alt_Port_Isol;
      mask prompts: Parameter1 "entity name"; Parameter2 "sampling time"; Parameter3 "project"; resources "input resources and state variables"; Parameter10 "Bring state variables to output"; codeupdate "update code from mask"
      mask help: This is a level-2 MATLAB file S-function which demonstrates CISIA entity
      mask DialogControl Container1 Prompt: All parameters
      mask Display: image('Icons/MobileUnit.png')
  Mobile_2 (148) : M-S-Function  FunctionName=cisia_msfun  Parameters=Parameter1, Parameter2, Parameter3, resources, Parameter10, codeupdate, step_received, step_computed, dynamic_computed, step_sended, id_entity, id_project, id_type, name_type, color  mask(S-function:msfcn_unit_delay){Parameter1='Mobile_2', Parameter2=1, Parameter3='ORO', resources=, Parameter10=off, codeupdate=off, step_received=|, step_computed=, dynamic_computed=, step_sended=|, id_entity=148, id_project=6, id_type=39, name_type=MobileUnit, color=#C9ABDB}
      mask step_received=|
      | Connection=max(Connection_init,R_CONN);
      | TLC_services=max(TLC_services_init,TLC_SERVICE);
      | TLC_services=mod(TLC_services,10);
      | TLC_revoke=floor(TLC_SERVICE/10);
      |
      | Service_Fault=max(abs(Consumed_Services.*TLC_services-Consumed_Services));
      | Redundancy_Fault=max(abs(Consumed_Services.*R_CONN-Consumed_Services));
      |
      | Alt_Serv_Fault=max(abs(Alternative_Services.*R_CONN-Alternative_Services));
      |
      | Alt_Rout_Fault=max(abs(Consumed_Services.*R_CONN-Consumed_Services));
      |
      | Port_Isolation=min(max(transpose([1 1 1 1 1 1 1 1 1 0]), CYBER_FAULT));
      |
      |
      | Operative_Level=(1-Mechanical_Fault)*max(max(R_CONN), 0.5)*(((1-Service_Fault)+(1-Redundancy_Fault)+(1-Port_Isolation))/3);
      |
      | Alt_Port_Isol=(1-Mechanical_Fault)*max(max(R_CONN), 0.5)*(((1-Service_Fault)+(1-Redundancy_Fault))/2);
      mask step_sended=|
      | MOBILE_QoS=Operative_Level;
      |
      |
      | ALT_SERVICES=1-Alt_Serv_Fault;
      | ALT_ROUTING=1-Alt_Rout_Fault;
      | ALT_PORT_ISOLATION=Alt_Port_Isol;
      mask prompts: Parameter1 "entity name"; Parameter2 "sampling time"; Parameter3 "project"; resources "input resources and state variables"; Parameter10 "Bring state variables to output"; codeupdate "update code from mask"
      mask help: This is a level-2 MATLAB file S-function which demonstrates CISIA entity
      mask DialogControl Container1 Prompt: All parameters
      mask Display: image('Icons/MobileUnit.png')
  Mux : Mux  Inputs=9
  Mux{1,3..5} (4 alike) : Mux  Inputs=3
  Nex_1 (3) : M-S-Function  FunctionName=cisia_msfun  Parameters=Parameter1, Parameter2, Parameter3, resources, Parameter10, codeupdate, step_received, step_computed, dynamic_computed, step_sended, id_entity, id_project, id_type, name_type, color  mask(S-function:msfcn_unit_delay){Parameter1='Nex_1', Parameter2=1, Parameter3='ORO', resources=, Parameter10=off, codeupdate=off, step_received=|, step_computed=, dynamic_computed=, step_sended=|, id_entity=3, id_project=6, id_type=2, name_type=Nexus93180Switch, color=#0072BD}
      mask step_received=|
      | Connection=max(Connection_init,TLC_CONN);
      |
      | TLC_services=max(TLC_services_init,TLC_SERVICE);
      | TLC_services=mod(TLC_services,10);
      | TLC_revoke=floor(TLC_SERVICE/10);
      |
      | Cyber_Fault=max(CYBER_FAULT, transpose([Dos_attack   MITM_attack Virus_Attack Port_Scan_Attack  BGP_hijacking BotNet_Attack Data_Corruption SW_Change Config_Change Port_Saturation]));
      |
      | Conn_Fault=max([Dos_attack  Mechanical_Fault  1-POWER 1-ROOM_QoS] );
      |
      | Operative_Level=(1-Conn_Fault)*max(max(TLC_services),0.5)*(1-0.5*max(Cyber_Fault));
      mask step_sended=|
      | TLC_CONN=Connection*(1-Conn_Fault);
      | TLC_SERVICE=TLC_services*(1-Conn_Fault)+10*TLC_revoke;
      |
      | Cyber_Transmitted=min(Cyber_Fault, transpose([0 0 1 0 1 1 0 0 0 1]));
      | CYBER_FAULT=Cyber_Transmitted*(1-Conn_Fault);
      |
      |
      | SWITCHING_QoS=Operative_Level;
      mask prompts: Parameter1 "entity name"; Parameter2 "sampling time"; Parameter3 "project"; resources "input resources and state variables"; Parameter10 "Bring state variables to output"; codeupdate "update code from mask"
      mask help: This is a level-2 MATLAB file S-function which demonstrates CISIA entity
      mask DialogControl Container1 Prompt: All parameters
      mask Display: image('Icons/Nexus93180Switch.png')
  Nex_2 (4) : M-S-Function  FunctionName=cisia_msfun  Parameters=Parameter1, Parameter2, Parameter3, resources, Parameter10, codeupdate, step_received, step_computed, dynamic_computed, step_sended, id_entity, id_project, id_type, name_type, color  mask(S-function:msfcn_unit_delay){Parameter1='Nex_2', Parameter2=1, Parameter3='ORO', resources=, Parameter10=off, codeupdate=off, step_received=|, step_computed=, dynamic_computed=, step_sended=|, id_entity=4, id_project=6, id_type=2, name_type=Nexus93180Switch, color=#0072BD}
      mask step_received=|
      | Connection=max(Connection_init,TLC_CONN);
      |
      | TLC_services=max(TLC_services_init,TLC_SERVICE);
      | TLC_services=mod(TLC_services,10);
      | TLC_revoke=floor(TLC_SERVICE/10);
      |
      | Cyber_Fault=max(CYBER_FAULT, transpose([Dos_attack   MITM_attack Virus_Attack Port_Scan_Attack  BGP_hijacking BotNet_Attack Data_Corruption SW_Change Config_Change Port_Saturation]));
      |
      | Conn_Fault=max([Dos_attack  Mechanical_Fault  1-POWER 1-ROOM_QoS] );
      |
      | Operative_Level=(1-Conn_Fault)*max(max(TLC_services),0.5)*(1-0.5*max(Cyber_Fault));
      mask step_sended=|
      | TLC_CONN=Connection*(1-Conn_Fault);
      | TLC_SERVICE=TLC_services*(1-Conn_Fault)+10*TLC_revoke;
      |
      | Cyber_Transmitted=min(Cyber_Fault, transpose([0 0 1 0 1 1 0 0 0 1]));
      | CYBER_FAULT=Cyber_Transmitted*(1-Conn_Fault);
      |
      |
      | SWITCHING_QoS=Operative_Level;
      mask prompts: Parameter1 "entity name"; Parameter2 "sampling time"; Parameter3 "project"; resources "input resources and state variables"; Parameter10 "Bring state variables to output"; codeupdate "update code from mask"
      mask help: This is a level-2 MATLAB file S-function which demonstrates CISIA entity
      mask DialogControl Container1 Prompt: All parameters
      mask Display: image('Icons/Nexus93180Switch.png')
  ONU_1 (55) : M-S-Function  FunctionName=cisia_msfun  Parameters=Parameter1, Parameter2, Parameter3, resources, Parameter10, codeupdate, step_received, step_computed, dynamic_computed, step_sended, id_entity, id_project, id_type, name_type, color  mask(S-function:msfcn_unit_delay){Parameter1='ONU_1', Parameter2=1, Parameter3='ORO', resources=, Parameter10=off, codeupdate=off, step_received=|, step_computed=, dynamic_computed=, step_sended=|, id_entity=55, id_project=6, id_type=12, name_type=ONU, color=#90DB5A}
      mask step_received=|
      | Connection=max(Connection_init,NGPON_CONN);
      | TLC_services=max(TLC_services_init,TLC_SERVICE);
      | TLC_services=mod(TLC_services,10);
      | TLC_revoke=floor(TLC_SERVICE/10);
      |
      | Cyber_Fault=max(CYBER_FAULT, transpose([Dos_attack   MITM_attack Virus_Attack Port_Scan_Attack  BGP_hijacking BotNet_Attack Data_Corruption SW_Change Config_Change Port_Saturation]));
      |
      | Conn_Fault=max([Dos_attack  Mechanical_Fault  1-POWER] );
      |
      | Service_Fault=max(abs(Consumed_Services.*TLC_services-Consumed_Services));
      | Redundancy_Fault=max(abs(Consumed_Services.*NGPON_CONN-Consumed_Services));
      |
      | Operative_Level=(1-Conn_Fault)*(1-0.5*max(Cyber_Fault))*(1-Service_Fault)*max(max(NGPON_CONN),0.5);
      |
      | %Operative_Level=(1-Conn_Fault)*max(max(TLC_services),0.5)*((2*(1-Service_Fault)+(1-Redundancy_Fault))/3);
      | % Il servizio utilizzato
      | %My_Service=max([(1-Service_Fault) (1-Redundancy_Fault)/2]);
      | %Operative_Level=(1-Conn_Fault);
      mask step_sended=|
      | TLC_SERVICE=TLC_services*(1-Conn_Fault)+10*TLC_revoke;
      | NGPON_CONN=Connection*(1-Conn_Fault);
      |
      | Cyber_Transmitted=min(Cyber_Fault, transpose([0 0 1 0 1 1 0 0 0 1]));
      | CYBER_FAULT=Cyber_Transmitted*(1-Conn_Fault);
      mask prompts: Parameter1 "entity name"; Parameter2 "sampling time"; Parameter3 "project"; resources "input resources and state variables"; Parameter10 "Bring state variables to output"; codeupdate "update code from mask"
      mask help: This is a level-2 MATLAB file S-function which demonstrates CISIA entity
      mask DialogControl Container1 Prompt: All parameters
      mask Display: disp('ONU')
  ONU_2 (58) : M-S-Function  FunctionName=cisia_msfun  Parameters=Parameter1, Parameter2, Parameter3, resources, Parameter10, codeupdate, step_received, step_computed, dynamic_computed, step_sended, id_entity, id_project, id_type, name_type, color  mask(S-function:msfcn_unit_delay){Parameter1='ONU_2', Parameter2=1, Parameter3='ORO', resources=, Parameter10=off, codeupdate=off, step_received=|, step_computed=, dynamic_computed=, step_sended=|, id_entity=58, id_project=6, id_type=12, name_type=ONU, color=#90DB5A}
      mask step_received=|
      | Connection=max(Connection_init,NGPON_CONN);
      | TLC_services=max(TLC_services_init,TLC_SERVICE);
      | TLC_services=mod(TLC_services,10);
      | TLC_revoke=floor(TLC_SERVICE/10);
      |
      | Cyber_Fault=max(CYBER_FAULT, transpose([Dos_attack   MITM_attack Virus_Attack Port_Scan_Attack  BGP_hijacking BotNet_Attack Data_Corruption SW_Change Config_Change Port_Saturation]));
      |
      | Conn_Fault=max([Dos_attack  Mechanical_Fault  1-POWER] );
      |
      | Service_Fault=max(abs(Consumed_Services.*TLC_services-Consumed_Services));
      | Redundancy_Fault=max(abs(Consumed_Services.*NGPON_CONN-Consumed_Services));
      |
      | Operative_Level=(1-Conn_Fault)*(1-0.5*max(Cyber_Fault))*(1-Service_Fault)*max(max(NGPON_CONN),0.5);
      |
      | %Operative_Level=(1-Conn_Fault)*max(max(TLC_services),0.5)*((2*(1-Service_Fault)+(1-Redundancy_Fault))/3);
      | % Il servizio utilizzato
      | %My_Service=max([(1-Service_Fault) (1-Redundancy_Fault)/2]);
      | %Operative_Level=(1-Conn_Fault);
      mask step_sended=|
      | TLC_SERVICE=TLC_services*(1-Conn_Fault)+10*TLC_revoke;
      | NGPON_CONN=Connection*(1-Conn_Fault);
      |
      | Cyber_Transmitted=min(Cyber_Fault, transpose([0 0 1 0 1 1 0 0 0 1]));
      | CYBER_FAULT=Cyber_Transmitted*(1-Conn_Fault);
      mask prompts: Parameter1 "entity name"; Parameter2 "sampling time"; Parameter3 "project"; resources "input resources and state variables"; Parameter10 "Bring state variables to output"; codeupdate "update code from mask"
      mask help: This is a level-2 MATLAB file S-function which demonstrates CISIA entity
      mask DialogControl Container1 Prompt: All parameters
      mask Display: disp('ONU')
  ONU_3 (282) : M-S-Function  FunctionName=cisia_msfun  Parameters=Parameter1, Parameter2, Parameter3, resources, Parameter10, codeupdate, step_received, step_computed, dynamic_computed, step_sended, id_entity, id_project, id_type, name_type, color  mask(S-function:msfcn_unit_delay){Parameter1='ONU_3', Parameter2=1, Parameter3='ORO', resources=, Parameter10=off, codeupdate=off, step_received=|, step_computed=, dynamic_computed=, step_sended=|, id_entity=282, id_project=6, id_type=12, name_type=ONU, color=#90DB5A}
      mask step_received=|
      | Connection=max(Connection_init,NGPON_CONN);
      | TLC_services=max(TLC_services_init,TLC_SERVICE);
      | TLC_services=mod(TLC_services,10);
      | TLC_revoke=floor(TLC_SERVICE/10);
      |
      | Cyber_Fault=max(CYBER_FAULT, transpose([Dos_attack   MITM_attack Virus_Attack Port_Scan_Attack  BGP_hijacking BotNet_Attack Data_Corruption SW_Change Config_Change Port_Saturation]));
      |
      | Conn_Fault=max([Dos_attack  Mechanical_Fault  1-POWER] );
      |
      | Service_Fault=max(abs(Consumed_Services.*TLC_services-Consumed_Services));
      | Redundancy_Fault=max(abs(Consumed_Services.*NGPON_CONN-Consumed_Services));
      |
      | Operative_Level=(1-Conn_Fault)*(1-0.5*max(Cyber_Fault))*(1-Service_Fault)*max(max(NGPON_CONN),0.5);
      |
      | %Operative_Level=(1-Conn_Fault)*max(max(TLC_services),0.5)*((2*(1-Service_Fault)+(1-Redundancy_Fault))/3);
      | % Il servizio utilizzato
      | %My_Service=max([(1-Service_Fault) (1-Redundancy_Fault)/2]);
      | %Operative_Level=(1-Conn_Fault);
      mask step_sended=|
      | TLC_SERVICE=TLC_services*(1-Conn_Fault)+10*TLC_revoke;
      | NGPON_CONN=Connection*(1-Conn_Fault);
      |
      | Cyber_Transmitted=min(Cyber_Fault, transpose([0 0 1 0 1 1 0 0 0 1]));
      | CYBER_FAULT=Cyber_Transmitted*(1-Conn_Fault);
      mask prompts: Parameter1 "entity name"; Parameter2 "sampling time"; Parameter3 "project"; resources "input resources and state variables"; Parameter10 "Bring state variables to output"; codeupdate "update code from mask"
      mask help: This is a level-2 MATLAB file S-function which demonstrates CISIA entity
      mask DialogControl Container1 Prompt: All parameters
      mask Display: disp('ONU')
  PowerGen_1 (46) : M-S-Function  FunctionName=cisia_msfun  Parameters=Parameter1, Parameter2, Parameter3, resources, Parameter10, codeupdate, step_received, step_computed, dynamic_computed, step_sended, id_entity, id_project, id_type, name_type, color  mask(S-function:msfcn_unit_delay){Parameter1='PowerGen_1', Parameter2=1, Parameter3='ORO', resources=, Parameter10=off, codeupdate=off, step_received=Operative_Level=1-Power_Fault;, step_computed=, dynamic_computed=, step_sended=POWER=Operative_Level;, id_entity=46, id_project=6, id_type=8, name_type=PowerSource, color=#84BD8C}
      mask prompts: Parameter1 "entity name"; Parameter2 "sampling time"; Parameter3 "project"; resources "input resources and state variables"; Parameter10 "Bring state variables to output"; codeupdate "update code from mask"
      mask help: This is a level-2 MATLAB file S-function which demonstrates CISIA entity
      mask DialogControl Container1 Prompt: All parameters
      mask Display: image('Icons/PowerSource.png')
  PowerGen_2 (47) : M-S-Function  FunctionName=cisia_msfun  Parameters=Parameter1, Parameter2, Parameter3, resources, Parameter10, codeupdate, step_received, step_computed, dynamic_computed, step_sended, id_entity, id_project, id_type, name_type, color  mask(S-function:msfcn_unit_delay){Parameter1='PowerGen_2', Parameter2=1, Parameter3='ORO', resources=, Parameter10=off, codeupdate=off, step_received=Operative_Level=1-Power_Fault;, step_computed=, dynamic_computed=, step_sended=POWER=Operative_Level;, id_entity=47, id_project=6, id_type=8, name_type=PowerSource, color=#84BD8C}
      mask prompts: Parameter1 "entity name"; Parameter2 "sampling time"; Parameter3 "project"; resources "input resources and state variables"; Parameter10 "Bring state variables to output"; codeupdate "update code from mask"
      mask help: This is a level-2 MATLAB file S-function which demonstrates CISIA entity
      mask DialogControl Container1 Prompt: All parameters
      mask Display: image('Icons/PowerSource.png')
  PowerGen_3 (157) : M-S-Function  FunctionName=cisia_msfun  Parameters=Parameter1, Parameter2, Parameter3, resources, Parameter10, codeupdate, step_received, step_computed, dynamic_computed, step_sended, id_entity, id_project, id_type, name_type, color  mask(S-function:msfcn_unit_delay){Parameter1='PowerGen_3', Parameter2=1, Parameter3='ORO', resources=, Parameter10=off, codeupdate=off, step_received=Operative_Level=1-Power_Fault;, step_computed=, dynamic_computed=, step_sended=POWER=Operative_Level;, id_entity=157, id_project=6, id_type=8, name_type=PowerSource, color=#84BD8C}
      mask prompts: Parameter1 "entity name"; Parameter2 "sampling time"; Parameter3 "project"; resources "input resources and state variables"; Parameter10 "Bring state variables to output"; codeupdate "update code from mask"
      mask help: This is a level-2 MATLAB file S-function which demonstrates CISIA entity
      mask DialogControl Container1 Prompt: All parameters
      mask Display: image('Icons/PowerSource.png')
  PowerGen_4 (214) : M-S-Function  FunctionName=cisia_msfun  Parameters=Parameter1, Parameter2, Parameter3, resources, Parameter10, codeupdate, step_received, step_computed, dynamic_computed, step_sended, id_entity, id_project, id_type, name_type, color  mask(S-function:msfcn_unit_delay){Parameter1='PowerGen_4', Parameter2=1, Parameter3='ORO', resources=, Parameter10=off, codeupdate=off, step_received=Operative_Level=1-Power_Fault;, step_computed=, dynamic_computed=, step_sended=POWER=Operative_Level;, id_entity=214, id_project=6, id_type=8, name_type=PowerSource, color=#84BD8C}
      mask prompts: Parameter1 "entity name"; Parameter2 "sampling time"; Parameter3 "project"; resources "input resources and state variables"; Parameter10 "Bring state variables to output"; codeupdate "update code from mask"
      mask help: This is a level-2 MATLAB file S-function which demonstrates CISIA entity
      mask DialogControl Container1 Prompt: All parameters
      mask Display: image('Icons/PowerSource.png')
  PowerGen_5 (236) : M-S-Function  FunctionName=cisia_msfun  Parameters=Parameter1, Parameter2, Parameter3, resources, Parameter10, codeupdate, step_received, step_computed, dynamic_computed, step_sended, id_entity, id_project, id_type, name_type, color  mask(S-function:msfcn_unit_delay){Parameter1='PowerGen_5', Parameter2=1, Parameter3='ORO', resources=, Parameter10=off, codeupdate=off, step_received=Operative_Level=1-Power_Fault;, step_computed=, dynamic_computed=, step_sended=POWER=Operative_Level;, id_entity=236, id_project=6, id_type=8, name_type=PowerSource, color=#84BD8C}
      mask prompts: Parameter1 "entity name"; Parameter2 "sampling time"; Parameter3 "project"; resources "input resources and state variables"; Parameter10 "Bring state variables to output"; codeupdate "update code from mask"
      mask help: This is a level-2 MATLAB file S-function which demonstrates CISIA entity
      mask DialogControl Container1 Prompt: All parameters
      mask Display: image('Icons/PowerSource.png')
  PowerGen_6 (245) : M-S-Function  FunctionName=cisia_msfun  Parameters=Parameter1, Parameter2, Parameter3, resources, Parameter10, codeupdate, step_received, step_computed, dynamic_computed, step_sended, id_entity, id_project, id_type, name_type, color  mask(S-function:msfcn_unit_delay){Parameter1='PowerGen_6', Parameter2=1, Parameter3='ORO', resources=, Parameter10=off, codeupdate=off, step_received=Operative_Level=1-Power_Fault;, step_computed=, dynamic_computed=, step_sended=POWER=Operative_Level;, id_entity=245, id_project=6, id_type=8, name_type=PowerSource, color=#84BD8C}
      mask prompts: Parameter1 "entity name"; Parameter2 "sampling time"; Parameter3 "project"; resources "input resources and state variables"; Parameter10 "Bring state variables to output"; codeupdate "update code from mask"
      mask help: This is a level-2 MATLAB file S-function which demonstrates CISIA entity
      mask DialogControl Container1 Prompt: All parameters
      mask Display: image('Icons/PowerSource.png')
  PowerGen_7 (260) : M-S-Function  FunctionName=cisia_msfun  Parameters=Parameter1, Parameter2, Parameter3, resources, Parameter10, codeupdate, step_received, step_computed, dynamic_computed, step_sended, id_entity, id_project, id_type, name_type, color  mask(S-function:msfcn_unit_delay){Parameter1='PowerGen_7', Parameter2=1, Parameter3='ORO', resources=, Parameter10=off, codeupdate=off, step_received=Operative_Level=1-Power_Fault;, step_computed=, dynamic_computed=, step_sended=POWER=Operative_Level;, id_entity=260, id_project=6, id_type=8, name_type=PowerSource, color=#84BD8C}
      mask prompts: Parameter1 "entity name"; Parameter2 "sampling time"; Parameter3 "project"; resources "input resources and state variables"; Parameter10 "Bring state variables to output"; codeupdate "update code from mask"
      mask help: This is a level-2 MATLAB file S-function which demonstrates CISIA entity
      mask DialogControl Container1 Prompt: All parameters
      mask Display: image('Icons/PowerSource.png')
  ROUTE_ORO_1 (24) : M-S-Function  FunctionName=cisia_msfun  Parameters=Parameter1, Parameter2, Parameter3, Parameter4, Parameter5, Parameter6, Parameter7  mask(S-function:msfcn_unit_delay){Parameter1='ROUTE_ORO_1', Parameter2=1, Parameter3='ORO', Parameter4=9, Parameter5=0, Parameter6=20, Parameter7=off}
      mask prompts: Parameter1 "entity name"; Parameter2 "sampling time"; Parameter3 "project"; Parameter4 "number of output links"; Parameter5 "default value for outputs"; Parameter6 "link dimension (unused))"; Parameter7 "select resource elements and output port from input"
      mask help: This is a level-2 MATLAB file S-function which demonstrates CISIA entity
      mask Display: disp('ROUTE')
  ROUTE_ORO_2 (25) : M-S-Function  FunctionName=cisia_msfun  Parameters=Parameter1, Parameter2, Parameter3, Parameter4, Parameter5, Parameter6, Parameter7  mask(S-function:msfcn_unit_delay){Parameter1='ROUTE_ORO_2', Parameter2=1, Parameter3='ORO', Parameter4=6, Parameter5=0, Parameter6=20, Parameter7=off}
      mask prompts: Parameter1 "entity name"; Parameter2 "sampling time"; Parameter3 "project"; Parameter4 "number of output links"; Parameter5 "default value for outputs"; Parameter6 "link dimension (unused))"; Parameter7 "select resource elements and output port from input"
      mask help: This is a level-2 MATLAB file S-function which demonstrates CISIA entity
      mask Display: disp('ROUTE')
  ROUTE_ORO_3 (26) : M-S-Function  FunctionName=cisia_msfun  Parameters=Parameter1, Parameter2, Parameter3, Parameter4, Parameter5, Parameter6, Parameter7  mask(S-function:msfcn_unit_delay){Parameter1='ROUTE_ORO_3', Parameter2=1, Parameter3='ORO', Parameter4=2, Parameter5=0, Parameter6=20, Parameter7=off}
      mask prompts: Parameter1 "entity name"; Parameter2 "sampling time"; Parameter3 "project"; Parameter4 "number of output links"; Parameter5 "default value for outputs"; Parameter6 "link dimension (unused))"; Parameter7 "select resource elements and output port from input"
      mask help: This is a level-2 MATLAB file S-function which demonstrates CISIA entity
      mask Display: disp('ROUTE')
  ROUTE_ORO_4 (27) : M-S-Function  FunctionName=cisia_msfun  Parameters=Parameter1, Parameter2, Parameter3, Parameter4, Parameter5, Parameter6, Parameter7  mask(S-function:msfcn_unit_delay){Parameter1='ROUTE_ORO_4', Parameter2=1, Parameter3='ORO', Parameter4=3, Parameter5=0, Parameter6=20, Parameter7=off}
      mask prompts: Parameter1 "entity name"; Parameter2 "sampling time"; Parameter3 "project"; Parameter4 "number of output links"; Parameter5 "default value for outputs"; Parameter6 "link dimension (unused))"; Parameter7 "select resource elements and output port from input"
      mask help: This is a level-2 MATLAB file S-function which demonstrates CISIA entity
      mask Display: disp('ROUTE')
  ROUTE_ORO_7 (38) : M-S-Function  FunctionName=cisia_msfun  Parameters=Parameter1, Parameter2, Parameter3, Parameter4, Parameter5, Parameter6, Parameter7  mask(S-function:msfcn_unit_delay){Parameter1='ROUTE_ORO_7', Parameter2=1, Parameter3='ORO', Parameter4=2, Parameter5=0, Parameter6=20, Parameter7=off}
      mask prompts: Parameter1 "entity name"; Parameter2 "sampling time"; Parameter3 "project"; Parameter4 "number of output links"; Parameter5 "default value for outputs"; Parameter6 "link dimension (unused))"; Parameter7 "select resource elements and output port from input"
      mask help: This is a level-2 MATLAB file S-function which demonstrates CISIA entity
      mask Display: disp('ROUTE')
  ROUTE_ORO_9 (40) : M-S-Function  FunctionName=cisia_msfun  Parameters=Parameter1, Parameter2, Parameter3, Parameter4, Parameter5, Parameter6, Parameter7  mask(S-function:msfcn_unit_delay){Parameter1='ROUTE_ORO_9', Parameter2=1, Parameter3='ORO', Parameter4=2, Parameter5=0, Parameter6=20, Parameter7=off}
      mask prompts: Parameter1 "entity name"; Parameter2 "sampling time"; Parameter3 "project"; Parameter4 "number of output links"; Parameter5 "default value for outputs"; Parameter6 "link dimension (unused))"; Parameter7 "select resource elements and output port from input"
      mask help: This is a level-2 MATLAB file S-function which demonstrates CISIA entity
      mask Display: disp('ROUTE')
  R_Wire_1 (98) : M-S-Function  FunctionName=cisia_msfun  Parameters=Parameter1, Parameter2, Parameter3, resources, Parameter10, codeupdate, step_received, step_computed, dynamic_computed, step_sended, id_entity, id_project, id_type, name_type, color  mask(S-function:msfcn_unit_delay){Parameter1='R_Wire_1', Parameter2=1, Parameter3='ORO', resources=, Parameter10=off, codeupdate=off, step_received=|, step_computed=, dynamic_computed=, step_sended=|, id_entity=98, id_project=6, id_type=21, name_type=Redundant_Wire, color=#038F03}
      mask step_received=|
      | Connection=max(Connection_init,TLC_CONN);
      | TLC_services=max(TLC_services_init,TLC_SERVICE);
      | TLC_services=mod(TLC_services,10);
      | TLC_revoke=floor(TLC_SERVICE/10);
      |
      | Cyber_Fault=CYBER_FAULT;
      |
      | Mechanical_Fault=max([Mechanical_Fault MECH_FAULT Mechanical_Fault_init]);
      |
      | %TLC_services=TLC_services.*(1-TLC_revoke);
      |
      | Operative_Level=1-Mechanical_Fault;
      mask step_sended=|
      | TLC_CONN=Connection*Operative_Level;
      | TLC_SERVICE=TLC_services*Operative_Level+10*TLC_revoke;
      | CYBER_FAULT=Cyber_Fault*Operative_Level;
      | MECH_FAULT=Mechanical_Fault;
      mask prompts: Parameter1 "entity name"; Parameter2 "sampling time"; Parameter3 "project"; resources "input resources and state variables"; Parameter10 "Bring state variables to output"; codeupdate "update code from mask"
      mask help: This is a level-2 MATLAB file S-function which demonstrates CISIA entity
      mask DialogControl Container1 Prompt: All parameters
      mask Display: disp('Redundant_Wire')
  R_Wire_1b (99) : M-S-Function  FunctionName=cisia_msfun  Parameters=Parameter1, Parameter2, Parameter3, resources, Parameter10, codeupdate, step_received, step_computed, dynamic_computed, step_sended, id_entity, id_project, id_type, name_type, color  mask(S-function:msfcn_unit_delay){Parameter1='R_Wire_1b', Parameter2=1, Parameter3='ORO', resources=, Parameter10=off, codeupdate=off, step_received=|, step_computed=, dynamic_computed=, step_sended=|, id_entity=99, id_project=6, id_type=21, name_type=Redundant_Wire, color=#038F03}
      mask step_received=|
      | Connection=max(Connection_init,TLC_CONN);
      | TLC_services=max(TLC_services_init,TLC_SERVICE);
      | TLC_services=mod(TLC_services,10);
      | TLC_revoke=floor(TLC_SERVICE/10);
      |
      | Cyber_Fault=CYBER_FAULT;
      |
      | Mechanical_Fault=max([Mechanical_Fault MECH_FAULT Mechanical_Fault_init]);
      |
      | %TLC_services=TLC_services.*(1-TLC_revoke);
      |
      | Operative_Level=1-Mechanical_Fault;
      mask step_sended=|
      | TLC_CONN=Connection*Operative_Level;
      | TLC_SERVICE=TLC_services*Operative_Level+10*TLC_revoke;
      | CYBER_FAULT=Cyber_Fault*Operative_Level;
      | MECH_FAULT=Mechanical_Fault;
      mask prompts: Parameter1 "entity name"; Parameter2 "sampling time"; Parameter3 "project"; resources "input resources and state variables"; Parameter10 "Bring state variables to output"; codeupdate "update code from mask"
      mask help: This is a level-2 MATLAB file S-function which demonstrates CISIA entity
      mask DialogControl Container1 Prompt: All parameters
      mask Display: disp('Redundant_Wire')
  Room_1 (51) : M-S-Function  FunctionName=cisia_msfun  Parameters=Parameter1, Parameter2, Parameter3, resources, Parameter10, codeupdate, step_received, step_computed, dynamic_computed, step_sended, id_entity, id_project, id_type, name_type, color  mask(S-function:msfcn_unit_delay){Parameter1='Room_1', Parameter2=1, Parameter3='ORO', resources=, Parameter10=off, codeupdate=off, step_received=|, step_computed=, dynamic_computed=, step_sended=ROOM_QoS=Operative_Level;, id_entity=51, id_project=6, id_type=9, name_type=Room, color=#EDB120}
      mask step_received=|
      | Physical_Fault=max([Power_Fault Flooding_Fault Fire_Fault Cooling_Fault 1-POWER]);
      |
      |
      | %Operative_Level=min([1-Power_Fault 1-Flooding_Fault  1-Fire_Fault  1-Cooling_Fault  POWER]);
      | %Operative_Level=Operative_Level*max((1-Unauthorized_Access),0.5);
      |
      | Operative_Level=(1-Physical_Fault)*(1-0.5*Unauthorized_Access);
      mask prompts: Parameter1 "entity name"; Parameter2 "sampling time"; Parameter3 "project"; resources "input resources and state variables"; Parameter10 "Bring state variables to output"; codeupdate "update code from mask"
      mask help: This is a level-2 MATLAB file S-function which demonstrates CISIA entity
      mask DialogControl Container1 Prompt: All parameters
      mask Display: image('Icons/Room.png')
  Room_2 (52) : M-S-Function  FunctionName=cisia_msfun  Parameters=Parameter1, Parameter2, Parameter3, resources, Parameter10, codeupdate, step_received, step_computed, dynamic_computed, step_sended, id_entity, id_project, id_type, name_type, color  mask(S-function:msfcn_unit_delay){Parameter1='Room_2', Parameter2=1, Parameter3='ORO', resources=, Parameter10=off, codeupdate=off, step_received=|, step_computed=, dynamic_computed=, step_sended=ROOM_QoS=Operative_Level;, id_entity=52, id_project=6, id_type=9, name_type=Room, color=#EDB120}
      mask step_received=|
      | Physical_Fault=max([Power_Fault Flooding_Fault Fire_Fault Cooling_Fault 1-POWER]);
      |
      |
      | %Operative_Level=min([1-Power_Fault 1-Flooding_Fault  1-Fire_Fault  1-Cooling_Fault  POWER]);
      | %Operative_Level=Operative_Level*max((1-Unauthorized_Access),0.5);
      |
      | Operative_Level=(1-Physical_Fault)*(1-0.5*Unauthorized_Access);
      mask prompts: Parameter1 "entity name"; Parameter2 "sampling time"; Parameter3 "project"; resources "input resources and state variables"; Parameter10 "Bring state variables to output"; codeupdate "update code from mask"
      mask help: This is a level-2 MATLAB file S-function which demonstrates CISIA entity
      mask DialogControl Container1 Prompt: All parameters
      mask Display: image('Icons/Room.png')
  Room_3 (200) : M-S-Function  FunctionName=cisia_msfun  Parameters=Parameter1, Parameter2, Parameter3, resources, Parameter10, codeupdate, step_received, step_computed, dynamic_computed, step_sended, id_entity, id_project, id_type, name_type, color  mask(S-function:msfcn_unit_delay){Parameter1='Room_3', Parameter2=1, Parameter3='ORO', resources=, Parameter10=off, codeupdate=off, step_received=|, step_computed=, dynamic_computed=, step_sended=ROOM_QoS=Operative_Level;, id_entity=200, id_project=6, id_type=9, name_type=Room, color=#EDB120}
      mask step_received=|
      | Physical_Fault=max([Power_Fault Flooding_Fault Fire_Fault Cooling_Fault 1-POWER]);
      |
      |
      | %Operative_Level=min([1-Power_Fault 1-Flooding_Fault  1-Fire_Fault  1-Cooling_Fault  POWER]);
      | %Operative_Level=Operative_Level*max((1-Unauthorized_Access),0.5);
      |
      | Operative_Level=(1-Physical_Fault)*(1-0.5*Unauthorized_Access);
      mask prompts: Parameter1 "entity name"; Parameter2 "sampling time"; Parameter3 "project"; resources "input resources and state variables"; Parameter10 "Bring state variables to output"; codeupdate "update code from mask"
      mask help: This is a level-2 MATLAB file S-function which demonstrates CISIA entity
      mask DialogControl Container1 Prompt: All parameters
      mask Display: image('Icons/Room.png')
  Room_4 (237) : M-S-Function  FunctionName=cisia_msfun  Parameters=Parameter1, Parameter2, Parameter3, resources, Parameter10, codeupdate, step_received, step_computed, dynamic_computed, step_sended, id_entity, id_project, id_type, name_type, color  mask(S-function:msfcn_unit_delay){Parameter1='Room_4', Parameter2=1, Parameter3='ORO', resources=, Parameter10=off, codeupdate=off, step_received=|, step_computed=, dynamic_computed=, step_sended=ROOM_QoS=Operative_Level;, id_entity=237, id_project=6, id_type=9, name_type=Room, color=#EDB120}
      mask step_received=|
      | Physical_Fault=max([Power_Fault Flooding_Fault Fire_Fault Cooling_Fault 1-POWER]);
      |
      |
      | %Operative_Level=min([1-Power_Fault 1-Flooding_Fault  1-Fire_Fault  1-Cooling_Fault  POWER]);
      | %Operative_Level=Operative_Level*max((1-Unauthorized_Access),0.5);
      |
      | Operative_Level=(1-Physical_Fault)*(1-0.5*Unauthorized_Access);
      mask prompts: Parameter1 "entity name"; Parameter2 "sampling time"; Parameter3 "project"; resources "input resources and state variables"; Parameter10 "Bring state variables to output"; codeupdate "update code from mask"
      mask help: This is a level-2 MATLAB file S-function which demonstrates CISIA entity
      mask DialogControl Container1 Prompt: All parameters
      mask Display: image('Icons/Room.png')
  Room_5 (240) : M-S-Function  FunctionName=cisia_msfun  Parameters=Parameter1, Parameter2, Parameter3, resources, Parameter10, codeupdate, step_received, step_computed, dynamic_computed, step_sended, id_entity, id_project, id_type, name_type, color  mask(S-function:msfcn_unit_delay){Parameter1='Room_5', Parameter2=1, Parameter3='ORO', resources=, Parameter10=off, codeupdate=off, step_received=|, step_computed=, dynamic_computed=, step_sended=ROOM_QoS=Operative_Level;, id_entity=240, id_project=6, id_type=9, name_type=Room, color=#EDB120}
      mask step_received=|
      | Physical_Fault=max([Power_Fault Flooding_Fault Fire_Fault Cooling_Fault 1-POWER]);
      |
      |
      | %Operative_Level=min([1-Power_Fault 1-Flooding_Fault  1-Fire_Fault  1-Cooling_Fault  POWER]);
      | %Operative_Level=Operative_Level*max((1-Unauthorized_Access),0.5);
      |
      | Operative_Level=(1-Physical_Fault)*(1-0.5*Unauthorized_Access);
      mask prompts: Parameter1 "entity name"; Parameter2 "sampling time"; Parameter3 "project"; resources "input resources and state variables"; Parameter10 "Bring state variables to output"; codeupdate "update code from mask"
      mask help: This is a level-2 MATLAB file S-function which demonstrates CISIA entity
      mask DialogControl Container1 Prompt: All parameters
      mask Display: image('Icons/Room.png')
  Room_6 (241) : M-S-Function  FunctionName=cisia_msfun  Parameters=Parameter1, Parameter2, Parameter3, resources, Parameter10, codeupdate, step_received, step_computed, dynamic_computed, step_sended, id_entity, id_project, id_type, name_type, color  mask(S-function:msfcn_unit_delay){Parameter1='Room_6', Parameter2=1, Parameter3='ORO', resources=, Parameter10=off, codeupdate=off, step_received=|, step_computed=, dynamic_computed=, step_sended=ROOM_QoS=Operative_Level;, id_entity=241, id_project=6, id_type=9, name_type=Room, color=#EDB120}
      mask step_received=|
      | Physical_Fault=max([Power_Fault Flooding_Fault Fire_Fault Cooling_Fault 1-POWER]);
      |
      |
      | %Operative_Level=min([1-Power_Fault 1-Flooding_Fault  1-Fire_Fault  1-Cooling_Fault  POWER]);
      | %Operative_Level=Operative_Level*max((1-Unauthorized_Access),0.5);
      |
      | Operative_Level=(1-Physical_Fault)*(1-0.5*Unauthorized_Access);
      mask prompts: Parameter1 "entity name"; Parameter2 "sampling time"; Parameter3 "project"; resources "input resources and state variables"; Parameter10 "Bring state variables to output"; codeupdate "update code from mask"
      mask help: This is a level-2 MATLAB file S-function which demonstrates CISIA entity
      mask DialogControl Container1 Prompt: All parameters
      mask Display: image('Icons/Room.png')
  Room_7 (252) : M-S-Function  FunctionName=cisia_msfun  Parameters=Parameter1, Parameter2, Parameter3, resources, Parameter10, codeupdate, step_received, step_computed, dynamic_computed, step_sended, id_entity, id_project, id_type, name_type, color  mask(S-function:msfcn_unit_delay){Parameter1='Room_7', Parameter2=1, Parameter3='ORO', resources=, Parameter10=off, codeupdate=off, step_received=|, step_computed=, dynamic_computed=, step_sended=ROOM_QoS=Operative_Level;, id_entity=252, id_project=6, id_type=9, name_type=Room, color=#EDB120}
      mask step_received=|
      | Physical_Fault=max([Power_Fault Flooding_Fault Fire_Fault Cooling_Fault 1-POWER]);
      |
      |
      | %Operative_Level=min([1-Power_Fault 1-Flooding_Fault  1-Fire_Fault  1-Cooling_Fault  POWER]);
      | %Operative_Level=Operative_Level*max((1-Unauthorized_Access),0.5);
      |
      | Operative_Level=(1-Physical_Fault)*(1-0.5*Unauthorized_Access);
      mask prompts: Parameter1 "entity name"; Parameter2 "sampling time"; Parameter3 "project"; resources "input resources and state variables"; Parameter10 "Bring state variables to output"; codeupdate "update code from mask"
      mask help: This is a level-2 MATLAB file S-function which demonstrates CISIA entity
      mask DialogControl Container1 Prompt: All parameters
      mask Display: image('Icons/Room.png')
  SAVE_1 (3) : M-S-Function  FunctionName=cisia_msfun  Parameters=Parameter1, Parameter2, Parameter3, Parameter4,Parameter5,Parameter6,Parameter7  mask(S-function:msfcn_unit_delay){Parameter1='SAVE_1', Parameter2=1, Parameter3='SistemiIoT', Parameter4=on, Parameter5=[0], Parameter6=[1], Parameter7=off}
      mask prompts: Parameter1 "entity name"; Parameter2 "sampling time"; Parameter3 "project"; Parameter4 "display bars"; Parameter5 "values"; Parameter6 "logic"; Parameter7 "display B/W"
      mask help: This is a level-2 MATLAB file S-function which demonstrates CISIA entity
      mask DialogControl Container3 Prompt: Display
      mask Display:
      | display=get_param(gcb, 'Parameter4');
      | greymap=get_param(gcb, 'Parameter7');
      | 
      | if strcmp(display,'on')
      | 
      |     val=str2num(get_param(gcb, 'Parameter5'));
      |     logic=str2num(get_param(gcb, 'Parameter6'));
      |     n=length(val);
      | 
      |     val2=val;
      |     l=length(logic);
      |     if l>0
      |         for i=1:l
      |             if logic(i)==-1
      |                 val2(i)=1-val2(i);
      |             end
      |         end
      |     end
      | 
      | 
      | 
      | 
      |     if strcmp(greymap,'on')
      |         val_r=round(val2*50)+1;
      |         colormap=gray(60);
      |         color2=[0 0 0];
      |     else
      |         val_r=round(val2*20)+1;
      |         colormap=hsv(60);
      |         color2=[0 0 1];
      |     end
      | 
      |     patch([0 0 n n], [0 -0.2 -0.2 0], [1 1 1]);
      | 
      |     for i=1:n
      |         color=colormap(val_r(i),:);
      |         patch([i-1 i-1 i i],[0 1 1 0],color)
      |         patch([i-1 i],[val(i) val(i)],color2)
      | 
      |     end
      | 
      |     for i=1:n
      |         patch([i i], [-0.2 1], [0 0 0]);
      |         text(i-0.5, -0.1, num2str(val(i)));
      |     end
      | 
      | 
      | else
      | 
      |     disp('SAVE');
      | 
      | end
  SAVE_2 (2) : M-S-Function  FunctionName=cisia_msfun  Parameters=Parameter1, Parameter2, Parameter3, Parameter4,Parameter5,Parameter6,Parameter7  mask(S-function:msfcn_unit_delay){Parameter1='SAVE_2', Parameter2=1, Parameter3='SistemiIoT', Parameter4=on, Parameter5=[0.11111], Parameter6=[1], Parameter7=off}
      mask prompts: Parameter1 "entity name"; Parameter2 "sampling time"; Parameter3 "project"; Parameter4 "display bars"; Parameter5 "values"; Parameter6 "logic"; Parameter7 "display B/W"
      mask help: This is a level-2 MATLAB file S-function which demonstrates CISIA entity
      mask DialogControl Container3 Prompt: Display
      mask Display:
      | display=get_param(gcb, 'Parameter4');
      | greymap=get_param(gcb, 'Parameter7');
      | 
      | if strcmp(display,'on')
      | 
      |     val=str2num(get_param(gcb, 'Parameter5'));
      |     logic=str2num(get_param(gcb, 'Parameter6'));
      |     n=length(val);
      | 
      |     val2=val;
      |     l=length(logic);
      |     if l>0
      |         for i=1:l
      |             if logic(i)==-1
      |                 val2(i)=1-val2(i);
      |             end
      |         end
      |     end
      | 
      | 
      | 
      | 
      |     if strcmp(greymap,'on')
      |         val_r=round(val2*50)+1;
      |         colormap=gray(60);
      |         color2=[0 0 0];
      |     else
      |         val_r=round(val2*20)+1;
      |         colormap=hsv(60);
      |         color2=[0 0 1];
      |     end
      | 
      |     patch([0 0 n n], [0 -0.2 -0.2 0], [1 1 1]);
      | 
      |     for i=1:n
      |         color=colormap(val_r(i),:);
      |         patch([i-1 i-1 i i],[0 1 1 0],color)
      |         patch([i-1 i],[val(i) val(i)],color2)
      | 
      |     end
      | 
      |     for i=1:n
      |         patch([i i], [-0.2 1], [0 0 0]);
      |         text(i-0.5, -0.1, num2str(val(i)));
      |     end
      | 
      | 
      | else
      | 
      |     disp('SAVE');
      | 
      | end
  SAVE_20 (20) : M-S-Function  FunctionName=cisia_msfun  Parameters=Parameter1, Parameter2, Parameter3, Parameter4,Parameter5,Parameter6,Parameter7  mask(S-function:msfcn_unit_delay){Parameter1='SAVE_20', Parameter2=1, Parameter3='SistemiIoT', Parameter4=on, Parameter5=[0], Parameter6=[1], Parameter7=off}
      mask prompts: Parameter1 "entity name"; Parameter2 "sampling time"; Parameter3 "project"; Parameter4 "display bars"; Parameter5 "values"; Parameter6 "logic"; Parameter7 "display B/W"
      mask help: This is a level-2 MATLAB file S-function which demonstrates CISIA entity
      mask DialogControl Container3 Prompt: Display
      mask Display:
      | display=get_param(gcb, 'Parameter4');
      | greymap=get_param(gcb, 'Parameter7');
      | 
      | if strcmp(display,'on')
      | 
      |     val=str2num(get_param(gcb, 'Parameter5'));
      |     logic=str2num(get_param(gcb, 'Parameter6'));
      |     n=length(val);
      | 
      |     val2=val;
      |     l=length(logic);
      |     if l>0
      |         for i=1:l
      |             if logic(i)==-1
      |                 val2(i)=1-val2(i);
      |             end
      |         end
      |     end
      | 
      | 
      | 
      | 
      |     if strcmp(greymap,'on')
      |         val_r=round(val2*50)+1;
      |         colormap=gray(60);
      |         color2=[0 0 0];
      |     else
      |         val_r=round(val2*20)+1;
      |         colormap=hsv(60);
      |         color2=[0 0 1];
      |     end
      | 
      |     patch([0 0 n n], [0 -0.2 -0.2 0], [1 1 1]);
      | 
      |     for i=1:n
      |         color=colormap(val_r(i),:);
      |         patch([i-1 i-1 i i],[0 1 1 0],color)
      |         patch([i-1 i],[val(i) val(i)],color2)
      | 
      |     end
      | 
      |     for i=1:n
      |         patch([i i], [-0.2 1], [0 0 0]);
      |         text(i-0.5, -0.1, num2str(val(i)));
      |     end
      | 
      | 
      | else
      | 
      |     disp('SAVE');
      | 
      | end
  SAVE_21 (21) : M-S-Function  FunctionName=cisia_msfun  Parameters=Parameter1, Parameter2, Parameter3, Parameter4,Parameter5,Parameter6,Parameter7  mask(S-function:msfcn_unit_delay){Parameter1='SAVE_21', Parameter2=1, Parameter3='SistemiIoT', Parameter4=on, Parameter5=[0], Parameter6=[1], Parameter7=off}
      mask prompts: Parameter1 "entity name"; Parameter2 "sampling time"; Parameter3 "project"; Parameter4 "display bars"; Parameter5 "values"; Parameter6 "logic"; Parameter7 "display B/W"
      mask help: This is a level-2 MATLAB file S-function which demonstrates CISIA entity
      mask DialogControl Container3 Prompt: Display
      mask Display:
      | display=get_param(gcb, 'Parameter4');
      | greymap=get_param(gcb, 'Parameter7');
      | 
      | if strcmp(display,'on')
      | 
      |     val=str2num(get_param(gcb, 'Parameter5'));
      |     logic=str2num(get_param(gcb, 'Parameter6'));
      |     n=length(val);
      | 
      |     val2=val;
      |     l=length(logic);
      |     if l>0
      |         for i=1:l
      |             if logic(i)==-1
      |                 val2(i)=1-val2(i);
      |             end
      |         end
      |     end
      | 
      | 
      | 
      | 
      |     if strcmp(greymap,'on')
      |         val_r=round(val2*50)+1;
      |         colormap=gray(60);
      |         color2=[0 0 0];
      |     else
      |         val_r=round(val2*20)+1;
      |         colormap=hsv(60);
      |         color2=[0 0 1];
      |     end
      | 
      |     patch([0 0 n n], [0 -0.2 -0.2 0], [1 1 1]);
      | 
      |     for i=1:n
      |         color=colormap(val_r(i),:);
      |         patch([i-1 i-1 i i],[0 1 1 0],color)
      |         patch([i-1 i],[val(i) val(i)],color2)
      | 
      |     end
      | 
      |     for i=1:n
      |         patch([i i], [-0.2 1], [0 0 0]);
      |         text(i-0.5, -0.1, num2str(val(i)));
      |     end
      | 
      | 
      | else
      | 
      |     disp('SAVE');
      | 
      | end
  SAVE_22 (22) : M-S-Function  FunctionName=cisia_msfun  Parameters=Parameter1, Parameter2, Parameter3, Parameter4,Parameter5,Parameter6,Parameter7  mask(S-function:msfcn_unit_delay){Parameter1='SAVE_22', Parameter2=1, Parameter3='SistemiIoT', Parameter4=on, Parameter5=[0], Parameter6=[1], Parameter7=off}
      mask prompts: Parameter1 "entity name"; Parameter2 "sampling time"; Parameter3 "project"; Parameter4 "display bars"; Parameter5 "values"; Parameter6 "logic"; Parameter7 "display B/W"
      mask help: This is a level-2 MATLAB file S-function which demonstrates CISIA entity
      mask DialogControl Container3 Prompt: Display
      mask Display:
      | display=get_param(gcb, 'Parameter4');
      | greymap=get_param(gcb, 'Parameter7');
      | 
      | if strcmp(display,'on')
      | 
      |     val=str2num(get_param(gcb, 'Parameter5'));
      |     logic=str2num(get_param(gcb, 'Parameter6'));
      |     n=length(val);
      | 
      |     val2=val;
      |     l=length(logic);
      |     if l>0
      |         for i=1:l
      |             if logic(i)==-1
      |                 val2(i)=1-val2(i);
      |             end
      |         end
      |     end
      | 
      | 
      | 
      | 
      |     if strcmp(greymap,'on')
      |         val_r=round(val2*50)+1;
      |         colormap=gray(60);
      |         color2=[0 0 0];
      |     else
      |         val_r=round(val2*20)+1;
      |         colormap=hsv(60);
      |         color2=[0 0 1];
      |     end
      | 
      |     patch([0 0 n n], [0 -0.2 -0.2 0], [1 1 1]);
      | 
      |     for i=1:n
      |         color=colormap(val_r(i),:);
      |         patch([i-1 i-1 i i],[0 1 1 0],color)
      |         patch([i-1 i],[val(i) val(i)],color2)
      | 
      |     end
      | 
      |     for i=1:n
      |         patch([i i], [-0.2 1], [0 0 0]);
      |         text(i-0.5, -0.1, num2str(val(i)));
      |     end
      | 
      | 
      | else
      | 
      |     disp('SAVE');
      | 
      | end
  SAVE_23 (23) : M-S-Function  FunctionName=cisia_msfun  Parameters=Parameter1, Parameter2, Parameter3, Parameter4,Parameter5,Parameter6,Parameter7  mask(S-function:msfcn_unit_delay){Parameter1='SAVE_23', Parameter2=1, Parameter3='SistemiIoT', Parameter4=on, Parameter5=[0], Parameter6=[1], Parameter7=off}
      mask prompts: Parameter1 "entity name"; Parameter2 "sampling time"; Parameter3 "project"; Parameter4 "display bars"; Parameter5 "values"; Parameter6 "logic"; Parameter7 "display B/W"
      mask help: This is a level-2 MATLAB file S-function which demonstrates CISIA entity
      mask DialogControl Container3 Prompt: Display
      mask Display:
      | display=get_param(gcb, 'Parameter4');
      | greymap=get_param(gcb, 'Parameter7');
      | 
      | if strcmp(display,'on')
      | 
      |     val=str2num(get_param(gcb, 'Parameter5'));
      |     logic=str2num(get_param(gcb, 'Parameter6'));
      |     n=length(val);
      | 
      |     val2=val;
      |     l=length(logic);
      |     if l>0
      |         for i=1:l
      |             if logic(i)==-1
      |                 val2(i)=1-val2(i);
      |             end
      |         end
      |     end
      | 
      | 
      | 
      | 
      |     if strcmp(greymap,'on')
      |         val_r=round(val2*50)+1;
      |         colormap=gray(60);
      |         color2=[0 0 0];
      |     else
      |         val_r=round(val2*20)+1;
      |         colormap=hsv(60);
      |         color2=[0 0 1];
      |     end
      | 
      |     patch([0 0 n n], [0 -0.2 -0.2 0], [1 1 1]);
      | 
      |     for i=1:n
      |         color=colormap(val_r(i),:);
      |         patch([i-1 i-1 i i],[0 1 1 0],color)
      |         patch([i-1 i],[val(i) val(i)],color2)
      | 
      |     end
      | 
      |     for i=1:n
      |         patch([i i], [-0.2 1], [0 0 0]);
      |         text(i-0.5, -0.1, num2str(val(i)));
      |     end
      | 
      | 
      | else
      | 
      |     disp('SAVE');
      | 
      | end
  SAVE_3 (3) : M-S-Function  FunctionName=cisia_msfun  Parameters=Parameter1, Parameter2, Parameter3, Parameter4,Parameter5,Parameter6,Parameter7  mask(S-function:msfcn_unit_delay){Parameter1='SAVE_3', Parameter2=1, Parameter3='SistemiIoT', Parameter4=on, Parameter5=[0], Parameter6=[1], Parameter7=off}
      mask prompts: Parameter1 "entity name"; Parameter2 "sampling time"; Parameter3 "project"; Parameter4 "display bars"; Parameter5 "values"; Parameter6 "logic"; Parameter7 "display B/W"
      mask help: This is a level-2 MATLAB file S-function which demonstrates CISIA entity
      mask DialogControl Container3 Prompt: Display
      mask Display:
      | display=get_param(gcb, 'Parameter4');
      | greymap=get_param(gcb, 'Parameter7');
      | 
      | if strcmp(display,'on')
      | 
      |     val=str2num(get_param(gcb, 'Parameter5'));
      |     logic=str2num(get_param(gcb, 'Parameter6'));
      |     n=length(val);
      | 
      |     val2=val;
      |     l=length(logic);
      |     if l>0
      |         for i=1:l
      |             if logic(i)==-1
      |                 val2(i)=1-val2(i);
      |             end
      |         end
      |     end
      | 
      | 
      | 
      | 
      |     if strcmp(greymap,'on')
      |         val_r=round(val2*50)+1;
      |         colormap=gray(60);
      |         color2=[0 0 0];
      |     else
      |         val_r=round(val2*20)+1;
      |         colormap=hsv(60);
      |         color2=[0 0 1];
      |     end
      | 
      |     patch([0 0 n n], [0 -0.2 -0.2 0], [1 1 1]);
      | 
      |     for i=1:n
      |         color=colormap(val_r(i),:);
      |         patch([i-1 i-1 i i],[0 1 1 0],color)
      |         patch([i-1 i],[val(i) val(i)],color2)
      | 
      |     end
      | 
      |     for i=1:n
      |         patch([i i], [-0.2 1], [0 0 0]);
      |         text(i-0.5, -0.1, num2str(val(i)));
      |     end
      | 
      | 
      | else
      | 
      |     disp('SAVE');
      | 
      | end
  SAVE_4 (4) : M-S-Function  FunctionName=cisia_msfun  Parameters=Parameter1, Parameter2, Parameter3, Parameter4,Parameter5,Parameter6,Parameter7  mask(S-function:msfcn_unit_delay){Parameter1='SAVE_4', Parameter2=1, Parameter3='SistemiIoT', Parameter4=on, Parameter5=[0], Parameter6=[1], Parameter7=off}
      mask prompts: Parameter1 "entity name"; Parameter2 "sampling time"; Parameter3 "project"; Parameter4 "display bars"; Parameter5 "values"; Parameter6 "logic"; Parameter7 "display B/W"
      mask help: This is a level-2 MATLAB file S-function which demonstrates CISIA entity
      mask DialogControl Container3 Prompt: Display
      mask Display:
      | display=get_param(gcb, 'Parameter4');
      | greymap=get_param(gcb, 'Parameter7');
      | 
      | if strcmp(display,'on')
      | 
      |     val=str2num(get_param(gcb, 'Parameter5'));
      |     logic=str2num(get_param(gcb, 'Parameter6'));
      |     n=length(val);
      | 
      |     val2=val;
      |     l=length(logic);
      |     if l>0
      |         for i=1:l
      |             if logic(i)==-1
      |                 val2(i)=1-val2(i);
      |             end
      |         end
      |     end
      | 
      | 
      | 
      | 
      |     if strcmp(greymap,'on')
      |         val_r=round(val2*50)+1;
      |         colormap=gray(60);
      |         color2=[0 0 0];
      |     else
      |         val_r=round(val2*20)+1;
      |         colormap=hsv(60);
      |         color2=[0 0 1];
      |     end
      | 
      |     patch([0 0 n n], [0 -0.2 -0.2 0], [1 1 1]);
      | 
      |     for i=1:n
      |         color=colormap(val_r(i),:);
      |         patch([i-1 i-1 i i],[0 1 1 0],color)
      |         patch([i-1 i],[val(i) val(i)],color2)
      | 
      |     end
      | 
      |     for i=1:n
      |         patch([i i], [-0.2 1], [0 0 0]);
      |         text(i-0.5, -0.1, num2str(val(i)));
      |     end
      | 
      | 
      | else
      | 
      |     disp('SAVE');
      | 
      | end
  SAVE_5 (5) : M-S-Function  FunctionName=cisia_msfun  Parameters=Parameter1, Parameter2, Parameter3, Parameter4,Parameter5,Parameter6,Parameter7  mask(S-function:msfcn_unit_delay){Parameter1='SAVE_5', Parameter2=1, Parameter3='SistemiIoT', Parameter4=on, Parameter5=[0], Parameter6=[1], Parameter7=off}
      mask prompts: Parameter1 "entity name"; Parameter2 "sampling time"; Parameter3 "project"; Parameter4 "display bars"; Parameter5 "values"; Parameter6 "logic"; Parameter7 "display B/W"
      mask help: This is a level-2 MATLAB file S-function which demonstrates CISIA entity
      mask DialogControl Container3 Prompt: Display
      mask Display:
      | display=get_param(gcb, 'Parameter4');
      | greymap=get_param(gcb, 'Parameter7');
      | 
      | if strcmp(display,'on')
      | 
      |     val=str2num(get_param(gcb, 'Parameter5'));
      |     logic=str2num(get_param(gcb, 'Parameter6'));
      |     n=length(val);
      | 
      |     val2=val;
      |     l=length(logic);
      |     if l>0
      |         for i=1:l
      |             if logic(i)==-1
      |                 val2(i)=1-val2(i);
      |             end
      |         end
      |     end
      | 
      | 
      | 
      | 
      |     if strcmp(greymap,'on')
      |         val_r=round(val2*50)+1;
      |         colormap=gray(60);
      |         color2=[0 0 0];
      |     else
      |         val_r=round(val2*20)+1;
      |         colormap=hsv(60);
      |         color2=[0 0 1];
      |     end
      | 
      |     patch([0 0 n n], [0 -0.2 -0.2 0], [1 1 1]);
      | 
      |     for i=1:n
      |         color=colormap(val_r(i),:);
      |         patch([i-1 i-1 i i],[0 1 1 0],color)
      |         patch([i-1 i],[val(i) val(i)],color2)
      | 
      |     end
      | 
      |     for i=1:n
      |         patch([i i], [-0.2 1], [0 0 0]);
      |         text(i-0.5, -0.1, num2str(val(i)));
      |     end
      | 
      | 
      | else
      | 
      |     disp('SAVE');
      | 
      | end
  SAVE_6 (6) : M-S-Function  FunctionName=cisia_msfun  Parameters=Parameter1, Parameter2, Parameter3, Parameter4,Parameter5,Parameter6,Parameter7  mask(S-function:msfcn_unit_delay){Parameter1='SAVE_6', Parameter2=1, Parameter3='SistemiIoT', Parameter4=on, Parameter5=[0], Parameter6=[1], Parameter7=off}
      mask prompts: Parameter1 "entity name"; Parameter2 "sampling time"; Parameter3 "project"; Parameter4 "display bars"; Parameter5 "values"; Parameter6 "logic"; Parameter7 "display B/W"
      mask help: This is a level-2 MATLAB file S-function which demonstrates CISIA entity
      mask DialogControl Container3 Prompt: Display
      mask Display:
      | display=get_param(gcb, 'Parameter4');
      | greymap=get_param(gcb, 'Parameter7');
      | 
      | if strcmp(display,'on')
      | 
      |     val=str2num(get_param(gcb, 'Parameter5'));
      |     logic=str2num(get_param(gcb, 'Parameter6'));
      |     n=length(val);
      | 
      |     val2=val;
      |     l=length(logic);
      |     if l>0
      |         for i=1:l
      |             if logic(i)==-1
      |                 val2(i)=1-val2(i);
      |             end
      |         end
      |     end
      | 
      | 
      | 
      | 
      |     if strcmp(greymap,'on')
      |         val_r=round(val2*50)+1;
      |         colormap=gray(60);
      |         color2=[0 0 0];
      |     else
      |         val_r=round(val2*20)+1;
      |         colormap=hsv(60);
      |         color2=[0 0 1];
      |     end
      | 
      |     patch([0 0 n n], [0 -0.2 -0.2 0], [1 1 1]);
      | 
      |     for i=1:n
      |         color=colormap(val_r(i),:);
      |         patch([i-1 i-1 i i],[0 1 1 0],color)
      |         patch([i-1 i],[val(i) val(i)],color2)
      | 
      |     end
      | 
      |     for i=1:n
      |         patch([i i], [-0.2 1], [0 0 0]);
      |         text(i-0.5, -0.1, num2str(val(i)));
      |     end
      | 
      | 
      | else
      | 
      |     disp('SAVE');
      | 
      | end
  SAVE_7 (7) : M-S-Function  FunctionName=cisia_msfun  Parameters=Parameter1, Parameter2, Parameter3, Parameter4,Parameter5,Parameter6,Parameter7  mask(S-function:msfcn_unit_delay){Parameter1='SAVE_7', Parameter2=1, Parameter3='SistemiIoT', Parameter4=on, Parameter5=[0.5], Parameter6=[1], Parameter7=off}
      mask prompts: Parameter1 "entity name"; Parameter2 "sampling time"; Parameter3 "project"; Parameter4 "display bars"; Parameter5 "values"; Parameter6 "logic"; Parameter7 "display B/W"
      mask help: This is a level-2 MATLAB file S-function which demonstrates CISIA entity
      mask DialogControl Container3 Prompt: Display
      mask Display:
      | display=get_param(gcb, 'Parameter4');
      | greymap=get_param(gcb, 'Parameter7');
      | 
      | if strcmp(display,'on')
      | 
      |     val=str2num(get_param(gcb, 'Parameter5'));
      |     logic=str2num(get_param(gcb, 'Parameter6'));
      |     n=length(val);
      | 
      |     val2=val;
      |     l=length(logic);
      |     if l>0
      |         for i=1:l
      |             if logic(i)==-1
      |                 val2(i)=1-val2(i);
      |             end
      |         end
      |     end
      | 
      | 
      | 
      | 
      |     if strcmp(greymap,'on')
      |         val_r=round(val2*50)+1;
      |         colormap=gray(60);
      |         color2=[0 0 0];
      |     else
      |         val_r=round(val2*20)+1;
      |         colormap=hsv(60);
      |         color2=[0 0 1];
      |     end
      | 
      |     patch([0 0 n n], [0 -0.2 -0.2 0], [1 1 1]);
      | 
      |     for i=1:n
      |         color=colormap(val_r(i),:);
      |         patch([i-1 i-1 i i],[0 1 1 0],color)
      |         patch([i-1 i],[val(i) val(i)],color2)
      | 
      |     end
      | 
      |     for i=1:n
      |         patch([i i], [-0.2 1], [0 0 0]);
      |         text(i-0.5, -0.1, num2str(val(i)));
      |     end
      | 
      | 
      | else
      | 
      |     disp('SAVE');
      | 
      | end
  SAVE_8 (8) : M-S-Function  FunctionName=cisia_msfun  Parameters=Parameter1, Parameter2, Parameter3, Parameter4,Parameter5,Parameter6,Parameter7  mask(S-function:msfcn_unit_delay){Parameter1='SAVE_8', Parameter2=1, Parameter3='SistemiIoT', Parameter4=on, Parameter5=[0.2037], Parameter6=[1], Parameter7=off}
      mask prompts: Parameter1 "entity name"; Parameter2 "sampling time"; Parameter3 "project"; Parameter4 "display bars"; Parameter5 "values"; Parameter6 "logic"; Parameter7 "display B/W"
      mask help: This is a level-2 MATLAB file S-function which demonstrates CISIA entity
      mask DialogControl Container3 Prompt: Display
      mask Display:
      | display=get_param(gcb, 'Parameter4');
      | greymap=get_param(gcb, 'Parameter7');
      | 
      | if strcmp(display,'on')
      | 
      |     val=str2num(get_param(gcb, 'Parameter5'));
      |     logic=str2num(get_param(gcb, 'Parameter6'));
      |     n=length(val);
      | 
      |     val2=val;
      |     l=length(logic);
      |     if l>0
      |         for i=1:l
      |             if logic(i)==-1
      |                 val2(i)=1-val2(i);
      |             end
      |         end
      |     end
      | 
      | 
      | 
      | 
      |     if strcmp(greymap,'on')
      |         val_r=round(val2*50)+1;
      |         colormap=gray(60);
      |         color2=[0 0 0];
      |     else
      |         val_r=round(val2*20)+1;
      |         colormap=hsv(60);
      |         color2=[0 0 1];
      |     end
      | 
      |     patch([0 0 n n], [0 -0.2 -0.2 0], [1 1 1]);
      | 
      |     for i=1:n
      |         color=colormap(val_r(i),:);
      |         patch([i-1 i-1 i i],[0 1 1 0],color)
      |         patch([i-1 i],[val(i) val(i)],color2)
      | 
      |     end
      | 
      |     for i=1:n
      |         patch([i i], [-0.2 1], [0 0 0]);
      |         text(i-0.5, -0.1, num2str(val(i)));
      |     end
      | 
      | 
      | else
      | 
      |     disp('SAVE');
      | 
      | end
  Splitter_1 (54) : M-S-Function  FunctionName=cisia_msfun  Parameters=Parameter1, Parameter2, Parameter3, resources, Parameter10, codeupdate, step_received, step_computed, dynamic_computed, step_sended, id_entity, id_project, id_type, name_type, color  mask(S-function:msfcn_unit_delay){Parameter1='Splitter_1', Parameter2=1, Parameter3='ORO', resources=, Parameter10=off, codeupdate=off, step_received=|, step_computed=, dynamic_computed=, step_sended=|, id_entity=54, id_project=6, id_type=11, name_type=Splitter, color=#90DB5A}
      mask step_received=|
      | Connection=max(Connection_init,NGPON_CONN);
      | TLC_services=max(TLC_services_init,TLC_SERVICE);
      | TLC_services=mod(TLC_services,10);
      | TLC_revoke=floor(TLC_SERVICE/10);
      |
      | Cyber_Fault=max(CYBER_FAULT, transpose([Dos_attack   MITM_attack Virus_Attack Port_Scan_Attack  BGP_hijacking BotNet_Attack Data_Corruption SW_Change Config_Change Port_Saturation]));
      |
      | % Vale 1 in presenza di fault
      | Conn_Fault=max([Dos_attack  Mechanical_Fault] );
      |
      | Operative_Level=(1-Conn_Fault)*max(max(NGPON_CONN),0.5)*(1-0.5*max(Cyber_Fault)) ;
      mask step_sended=|
      | NGPON_IN=Connection;
      |
      | NGPON_CONN=Connection*(1-Conn_Fault);
      | TLC_SERVICE=TLC_services*(1-Conn_Fault)+10*TLC_revoke;
      |
      | Cyber_Transmitted=min(Cyber_Fault, transpose([0 0 1 0 1 1 0 0 0 1]));
      | CYBER_FAULT=Cyber_Transmitted*(1-Conn_Fault);
      |
      |
      | ROUTING_QoS=Operative_Level;
      mask prompts: Parameter1 "entity name"; Parameter2 "sampling time"; Parameter3 "project"; resources "input resources and state variables"; Parameter10 "Bring state variables to output"; codeupdate "update code from mask"
      mask help: This is a level-2 MATLAB file S-function which demonstrates CISIA entity
      mask DialogControl Container1 Prompt: All parameters
      mask Display: disp('Splitter')
  Subsystem : Subsystem
  Subsystem2 : Subsystem
  Subsystem3 : Subsystem
  Subsystem4 : Subsystem
  Subsystem5 : Subsystem
  Subsystem6 : Subsystem
  TLC_conn1 : MinMax  Function=max  Inputs=6
  TLC_conn11 : MinMax  Function=max  Inputs=2
  TLC_conn12 : MinMax  Function=max  Inputs=2
  TLC_conn2 : MinMax  Function=max  Inputs=6
  TLC_conn{3..5,8} (4 alike) : MinMax  Function=max  Inputs=4
  TLC_conn9 : MinMax  Function=max  Inputs=2
  TLC_service1 : MinMax  Function=max  Inputs=6
  TLC_service12 : MinMax  Function=max  Inputs=2
  TLC_service13 : MinMax  Function=max  Inputs=2
  TLC_service2 : MinMax  Function=max  Inputs=6
  TLC_service{3..5,8} (4 alike) : MinMax  Function=max  Inputs=4
  TLC_service9 : MinMax  Function=max  Inputs=2
  Wire_1 (1) : M-S-Function  FunctionName=cisia_msfun  Parameters=Parameter1, Parameter2, Parameter3, resources, Parameter10, codeupdate, step_received, step_computed, dynamic_computed, step_sended, id_entity, id_project, id_type, name_type, color  mask(S-function:msfcn_unit_delay){Parameter1='Wire_1', Parameter2=1, Parameter3='ORO', resources=, Parameter10=off, codeupdate=off, step_received=|, step_computed=, dynamic_computed=, step_sended=|, id_entity=1, id_project=6, id_type=1, name_type=Optical_Wire, color=#99CCFF}
      mask step_received=|
      | Connection=max(Connection_init,TLC_CONN);
      | TLC_services=max(TLC_services_init,TLC_SERVICE);
      | TLC_services=mod(TLC_services,10);
      | TLC_revoke=floor(TLC_SERVICE/10);
      |
      | Cyber_Fault=CYBER_FAULT;
      |
      | Mechanical_Fault=max([Mechanical_Fault MECH_FAULT Mechanical_Fault_init]);
      |
      | %TLC_services=TLC_services.*(1-TLC_revoke);
      |
      | Operative_Level=1-Mechanical_Fault;
      mask step_sended=|
      | TLC_CONN=Connection*Operative_Level;
      | TLC_SERVICE=TLC_services*Operative_Level+TLC_revoke*10;
      |
      |
      | CYBER_FAULT=Cyber_Fault*Operative_Level;
      | MECH_FAULT=Mechanical_Fault;
      mask prompts: Parameter1 "entity name"; Parameter2 "sampling time"; Parameter3 "project"; resources "input resources and state variables"; Parameter10 "Bring state variables to output"; codeupdate "update code from mask"
      mask help: This is a level-2 MATLAB file S-function which demonstrates CISIA entity
      mask DialogControl Container1 Prompt: All parameters
      mask Display: image('Icons/Optical_Wire.png')
  Wire_10 (30) : M-S-Function  FunctionName=cisia_msfun  Parameters=Parameter1, Parameter2, Parameter3, resources, Parameter10, codeupdate, step_received, step_computed, dynamic_computed, step_sended, id_entity, id_project, id_type, name_type, color  mask(S-function:msfcn_unit_delay){Parameter1='Wire_10', Parameter2=1, Parameter3='ORO', resources=, Parameter10=off, codeupdate=off, step_received=|, step_computed=, dynamic_computed=, step_sended=|, id_entity=30, id_project=6, id_type=1, name_type=Optical_Wire, color=#99CCFF}
      mask step_received=|
      | Connection=max(Connection_init,TLC_CONN);
      | TLC_services=max(TLC_services_init,TLC_SERVICE);
      | TLC_services=mod(TLC_services,10);
      | TLC_revoke=floor(TLC_SERVICE/10);
      |
      | Cyber_Fault=CYBER_FAULT;
      |
      | Mechanical_Fault=max([Mechanical_Fault MECH_FAULT Mechanical_Fault_init]);
      |
      | %TLC_services=TLC_services.*(1-TLC_revoke);
      |
      | Operative_Level=1-Mechanical_Fault;
      mask step_sended=|
      | TLC_CONN=Connection*Operative_Level;
      | TLC_SERVICE=TLC_services*Operative_Level+TLC_revoke*10;
      |
      |
      | CYBER_FAULT=Cyber_Fault*Operative_Level;
      | MECH_FAULT=Mechanical_Fault;
      mask prompts: Parameter1 "entity name"; Parameter2 "sampling time"; Parameter3 "project"; resources "input resources and state variables"; Parameter10 "Bring state variables to output"; codeupdate "update code from mask"
      mask help: This is a level-2 MATLAB file S-function which demonstrates CISIA entity
      mask DialogControl Container1 Prompt: All parameters
      mask Display: image('Icons/Optical_Wire.png')
  Wire_10b (31) : M-S-Function  FunctionName=cisia_msfun  Parameters=Parameter1, Parameter2, Parameter3, resources, Parameter10, codeupdate, step_received, step_computed, dynamic_computed, step_sended, id_entity, id_project, id_type, name_type, color  mask(S-function:msfcn_unit_delay){Parameter1='Wire_10b', Parameter2=1, Parameter3='ORO', resources=, Parameter10=off, codeupdate=off, step_received=|, step_computed=, dynamic_computed=, step_sended=|, id_entity=31, id_project=6, id_type=1, name_type=Optical_Wire, color=#99CCFF}
      mask step_received=|
      | Connection=max(Connection_init,TLC_CONN);
      | TLC_services=max(TLC_services_init,TLC_SERVICE);
      | TLC_services=mod(TLC_services,10);
      | TLC_revoke=floor(TLC_SERVICE/10);
      |
      | Cyber_Fault=CYBER_FAULT;
      |
      | Mechanical_Fault=max([Mechanical_Fault MECH_FAULT Mechanical_Fault_init]);
      |
      | %TLC_services=TLC_services.*(1-TLC_revoke);
      |
      | Operative_Level=1-Mechanical_Fault;
      mask step_sended=|
      | TLC_CONN=Connection*Operative_Level;
      | TLC_SERVICE=TLC_services*Operative_Level+TLC_revoke*10;
      |
      |
      | CYBER_FAULT=Cyber_Fault*Operative_Level;
      | MECH_FAULT=Mechanical_Fault;
      mask prompts: Parameter1 "entity name"; Parameter2 "sampling time"; Parameter3 "project"; resources "input resources and state variables"; Parameter10 "Bring state variables to output"; codeupdate "update code from mask"
      mask help: This is a level-2 MATLAB file S-function which demonstrates CISIA entity
      mask DialogControl Container1 Prompt: All parameters
      mask Display: image('Icons/Optical_Wire.png')
  Wire_12 (38) : M-S-Function  FunctionName=cisia_msfun  Parameters=Parameter1, Parameter2, Parameter3, resources, Parameter10, codeupdate, step_received, step_computed, dynamic_computed, step_sended, id_entity, id_project, id_type, name_type, color  mask(S-function:msfcn_unit_delay){Parameter1='Wire_12', Parameter2=1, Parameter3='ORO', resources=, Parameter10=off, codeupdate=off, step_received=|, step_computed=, dynamic_computed=, step_sended=|, id_entity=38, id_project=6, id_type=1, name_type=Optical_Wire, color=#99CCFF}
      mask step_received=|
      | Connection=max(Connection_init,TLC_CONN);
      | TLC_services=max(TLC_services_init,TLC_SERVICE);
      | TLC_services=mod(TLC_services,10);
      | TLC_revoke=floor(TLC_SERVICE/10);
      |
      | Cyber_Fault=CYBER_FAULT;
      |
      | Mechanical_Fault=max([Mechanical_Fault MECH_FAULT Mechanical_Fault_init]);
      |
      | %TLC_services=TLC_services.*(1-TLC_revoke);
      |
      | Operative_Level=1-Mechanical_Fault;
      mask step_sended=|
      | TLC_CONN=Connection*Operative_Level;
      | TLC_SERVICE=TLC_services*Operative_Level+TLC_revoke*10;
      |
      |
      | CYBER_FAULT=Cyber_Fault*Operative_Level;
      | MECH_FAULT=Mechanical_Fault;
      mask prompts: Parameter1 "entity name"; Parameter2 "sampling time"; Parameter3 "project"; resources "input resources and state variables"; Parameter10 "Bring state variables to output"; codeupdate "update code from mask"
      mask help: This is a level-2 MATLAB file S-function which demonstrates CISIA entity
      mask DialogControl Container1 Prompt: All parameters
      mask Display: image('Icons/Optical_Wire.png')
  Wire_12b (39) : M-S-Function  FunctionName=cisia_msfun  Parameters=Parameter1, Parameter2, Parameter3, resources, Parameter10, codeupdate, step_received, step_computed, dynamic_computed, step_sended, id_entity, id_project, id_type, name_type, color  mask(S-function:msfcn_unit_delay){Parameter1='Wire_12b', Parameter2=1, Parameter3='ORO', resources=, Parameter10=off, codeupdate=off, step_received=|, step_computed=, dynamic_computed=, step_sended=|, id_entity=39, id_project=6, id_type=1, name_type=Optical_Wire, color=#99CCFF}
      mask step_received=|
      | Connection=max(Connection_init,TLC_CONN);
      | TLC_services=max(TLC_services_init,TLC_SERVICE);
      | TLC_services=mod(TLC_services,10);
      | TLC_revoke=floor(TLC_SERVICE/10);
      |
      | Cyber_Fault=CYBER_FAULT;
      |
      | Mechanical_Fault=max([Mechanical_Fault MECH_FAULT Mechanical_Fault_init]);
      |
      | %TLC_services=TLC_services.*(1-TLC_revoke);
      |
      | Operative_Level=1-Mechanical_Fault;
      mask step_sended=|
      | TLC_CONN=Connection*Operative_Level;
      | TLC_SERVICE=TLC_services*Operative_Level+TLC_revoke*10;
      |
      |
      | CYBER_FAULT=Cyber_Fault*Operative_Level;
      | MECH_FAULT=Mechanical_Fault;
      mask prompts: Parameter1 "entity name"; Parameter2 "sampling time"; Parameter3 "project"; resources "input resources and state variables"; Parameter10 "Bring state variables to output"; codeupdate "update code from mask"
      mask help: This is a level-2 MATLAB file S-function which demonstrates CISIA entity
      mask DialogControl Container1 Prompt: All parameters
      mask Display: image('Icons/Optical_Wire.png')
  Wire_14 (42) : M-S-Function  FunctionName=cisia_msfun  Parameters=Parameter1, Parameter2, Parameter3, resources, Parameter10, codeupdate, step_received, step_computed, dynamic_computed, step_sended, id_entity, id_project, id_type, name_type, color  mask(S-function:msfcn_unit_delay){Parameter1='Wire_14', Parameter2=1, Parameter3='ORO', resources=, Parameter10=off, codeupdate=off, step_received=|, step_computed=, dynamic_computed=, step_sended=|, id_entity=42, id_project=6, id_type=1, name_type=Optical_Wire, color=#99CCFF}
      mask step_received=|
      | Connection=max(Connection_init,TLC_CONN);
      | TLC_services=max(TLC_services_init,TLC_SERVICE);
      | TLC_services=mod(TLC_services,10);
      | TLC_revoke=floor(TLC_SERVICE/10);
      |
      | Cyber_Fault=CYBER_FAULT;
      |
      | Mechanical_Fault=max([Mechanical_Fault MECH_FAULT Mechanical_Fault_init]);
      |
      | %TLC_services=TLC_services.*(1-TLC_revoke);
      |
      | Operative_Level=1-Mechanical_Fault;
      mask step_sended=|
      | TLC_CONN=Connection*Operative_Level;
      | TLC_SERVICE=TLC_services*Operative_Level+TLC_revoke*10;
      |
      |
      | CYBER_FAULT=Cyber_Fault*Operative_Level;
      | MECH_FAULT=Mechanical_Fault;
      mask prompts: Parameter1 "entity name"; Parameter2 "sampling time"; Parameter3 "project"; resources "input resources and state variables"; Parameter10 "Bring state variables to output"; codeupdate "update code from mask"
      mask help: This is a level-2 MATLAB file S-function which demonstrates CISIA entity
      mask DialogControl Container1 Prompt: All parameters
      mask Display: image('Icons/Optical_Wire.png')
  Wire_14b (43) : M-S-Function  FunctionName=cisia_msfun  Parameters=Parameter1, Parameter2, Parameter3, resources, Parameter10, codeupdate, step_received, step_computed, dynamic_computed, step_sended, id_entity, id_project, id_type, name_type, color  mask(S-function:msfcn_unit_delay){Parameter1='Wire_14b', Parameter2=1, Parameter3='ORO', resources=, Parameter10=off, codeupdate=off, step_received=|, step_computed=, dynamic_computed=, step_sended=|, id_entity=43, id_project=6, id_type=1, name_type=Optical_Wire, color=#99CCFF}
      mask step_received=|
      | Connection=max(Connection_init,TLC_CONN);
      | TLC_services=max(TLC_services_init,TLC_SERVICE);
      | TLC_services=mod(TLC_services,10);
      | TLC_revoke=floor(TLC_SERVICE/10);
      |
      | Cyber_Fault=CYBER_FAULT;
      |
      | Mechanical_Fault=max([Mechanical_Fault MECH_FAULT Mechanical_Fault_init]);
      |
      | %TLC_services=TLC_services.*(1-TLC_revoke);
      |
      | Operative_Level=1-Mechanical_Fault;
      mask step_sended=|
      | TLC_CONN=Connection*Operative_Level;
      | TLC_SERVICE=TLC_services*Operative_Level+TLC_revoke*10;
      |
      |
      | CYBER_FAULT=Cyber_Fault*Operative_Level;
      | MECH_FAULT=Mechanical_Fault;
      mask prompts: Parameter1 "entity name"; Parameter2 "sampling time"; Parameter3 "project"; resources "input resources and state variables"; Parameter10 "Bring state variables to output"; codeupdate "update code from mask"
      mask help: This is a level-2 MATLAB file S-function which demonstrates CISIA entity
      mask DialogControl Container1 Prompt: All parameters
      mask Display: image('Icons/Optical_Wire.png')
  Wire_15 (44) : M-S-Function  FunctionName=cisia_msfun  Parameters=Parameter1, Parameter2, Parameter3, resources, Parameter10, codeupdate, step_received, step_computed, dynamic_computed, step_sended, id_entity, id_project, id_type, name_type, color  mask(S-function:msfcn_unit_delay){Parameter1='Wire_15', Parameter2=1, Parameter3='ORO', resources=, Parameter10=off, codeupdate=off, step_received=|, step_computed=, dynamic_computed=, step_sended=|, id_entity=44, id_project=6, id_type=1, name_type=Optical_Wire, color=#99CCFF}
      mask step_received=|
      | Connection=max(Connection_init,TLC_CONN);
      | TLC_services=max(TLC_services_init,TLC_SERVICE);
      | TLC_services=mod(TLC_services,10);
      | TLC_revoke=floor(TLC_SERVICE/10);
      |
      | Cyber_Fault=CYBER_FAULT;
      |
      | Mechanical_Fault=max([Mechanical_Fault MECH_FAULT Mechanical_Fault_init]);
      |
      | %TLC_services=TLC_services.*(1-TLC_revoke);
      |
      | Operative_Level=1-Mechanical_Fault;
      mask step_sended=|
      | TLC_CONN=Connection*Operative_Level;
      | TLC_SERVICE=TLC_services*Operative_Level+TLC_revoke*10;
      |
      |
      | CYBER_FAULT=Cyber_Fault*Operative_Level;
      | MECH_FAULT=Mechanical_Fault;
      mask prompts: Parameter1 "entity name"; Parameter2 "sampling time"; Parameter3 "project"; resources "input resources and state variables"; Parameter10 "Bring state variables to output"; codeupdate "update code from mask"
      mask help: This is a level-2 MATLAB file S-function which demonstrates CISIA entity
      mask DialogControl Container1 Prompt: All parameters
      mask Display: image('Icons/Optical_Wire.png')
  Wire_15a (49) : M-S-Function  FunctionName=cisia_msfun  Parameters=Parameter1, Parameter2, Parameter3, resources, Parameter10, codeupdate, step_received, step_computed, dynamic_computed, step_sended, id_entity, id_project, id_type, name_type, color  mask(S-function:msfcn_unit_delay){Parameter1='Wire_15a', Parameter2=1, Parameter3='ORO', resources=, Parameter10=off, codeupdate=off, step_received=|, step_computed=, dynamic_computed=, step_sended=|, id_entity=49, id_project=6, id_type=1, name_type=Optical_Wire, color=#99CCFF}
      mask step_received=|
      | Connection=max(Connection_init,TLC_CONN);
      | TLC_services=max(TLC_services_init,TLC_SERVICE);
      | TLC_services=mod(TLC_services,10);
      | TLC_revoke=floor(TLC_SERVICE/10);
      |
      | Cyber_Fault=CYBER_FAULT;
      |
      | Mechanical_Fault=max([Mechanical_Fault MECH_FAULT Mechanical_Fault_init]);
      |
      | %TLC_services=TLC_services.*(1-TLC_revoke);
      |
      | Operative_Level=1-Mechanical_Fault;
      mask step_sended=|
      | TLC_CONN=Connection*Operative_Level;
      | TLC_SERVICE=TLC_services*Operative_Level+TLC_revoke*10;
      |
      |
      | CYBER_FAULT=Cyber_Fault*Operative_Level;
      | MECH_FAULT=Mechanical_Fault;
      mask prompts: Parameter1 "entity name"; Parameter2 "sampling time"; Parameter3 "project"; resources "input resources and state variables"; Parameter10 "Bring state variables to output"; codeupdate "update code from mask"
      mask help: This is a level-2 MATLAB file S-function which demonstrates CISIA entity
      mask DialogControl Container1 Prompt: All parameters
      mask Display: image('Icons/Optical_Wire.png')
  Wire_1b (96) : M-S-Function  FunctionName=cisia_msfun  Parameters=Parameter1, Parameter2, Parameter3, resources, Parameter10, codeupdate, step_received, step_computed, dynamic_computed, step_sended, id_entity, id_project, id_type, name_type, color  mask(S-function:msfcn_unit_delay){Parameter1='Wire_1b', Parameter2=1, Parameter3='ORO', resources=, Parameter10=off, codeupdate=off, step_received=|, step_computed=, dynamic_computed=, step_sended=|, id_entity=96, id_project=6, id_type=1, name_type=Optical_Wire, color=#99CCFF}
      mask step_received=|
      | Connection=max(Connection_init,TLC_CONN);
      | TLC_services=max(TLC_services_init,TLC_SERVICE);
      | TLC_services=mod(TLC_services,10);
      | TLC_revoke=floor(TLC_SERVICE/10);
      |
      | Cyber_Fault=CYBER_FAULT;
      |
      | Mechanical_Fault=max([Mechanical_Fault MECH_FAULT Mechanical_Fault_init]);
      |
      | %TLC_services=TLC_services.*(1-TLC_revoke);
      |
      | Operative_Level=1-Mechanical_Fault;
      mask step_sended=|
      | TLC_CONN=Connection*Operative_Level;
      | TLC_SERVICE=TLC_services*Operative_Level+TLC_revoke*10;
      |
      |
      | CYBER_FAULT=Cyber_Fault*Operative_Level;
      | MECH_FAULT=Mechanical_Fault;
      mask prompts: Parameter1 "entity name"; Parameter2 "sampling time"; Parameter3 "project"; resources "input resources and state variables"; Parameter10 "Bring state variables to output"; codeupdate "update code from mask"
      mask help: This is a level-2 MATLAB file S-function which demonstrates CISIA entity
      mask DialogControl Container1 Prompt: All parameters
      mask Display: image('Icons/Optical_Wire.png')
  Wire_2 (2) : M-S-Function  FunctionName=cisia_msfun  Parameters=Parameter1, Parameter2, Parameter3, resources, Parameter10, codeupdate, step_received, step_computed, dynamic_computed, step_sended, id_entity, id_project, id_type, name_type, color  mask(S-function:msfcn_unit_delay){Parameter1='Wire_2', Parameter2=1, Parameter3='ORO', resources=, Parameter10=off, codeupdate=off, step_received=|, step_computed=, dynamic_computed=, step_sended=|, id_entity=2, id_project=6, id_type=1, name_type=Optical_Wire, color=#99CCFF}
      mask step_received=|
      | Connection=max(Connection_init,TLC_CONN);
      | TLC_services=max(TLC_services_init,TLC_SERVICE);
      | TLC_services=mod(TLC_services,10);
      | TLC_revoke=floor(TLC_SERVICE/10);
      |
      | Cyber_Fault=CYBER_FAULT;
      |
      | Mechanical_Fault=max([Mechanical_Fault MECH_FAULT Mechanical_Fault_init]);
      |
      | %TLC_services=TLC_services.*(1-TLC_revoke);
      |
      | Operative_Level=1-Mechanical_Fault;
      mask step_sended=|
      | TLC_CONN=Connection*Operative_Level;
      | TLC_SERVICE=TLC_services*Operative_Level+TLC_revoke*10;
      |
      |
      | CYBER_FAULT=Cyber_Fault*Operative_Level;
      | MECH_FAULT=Mechanical_Fault;
      mask prompts: Parameter1 "entity name"; Parameter2 "sampling time"; Parameter3 "project"; resources "input resources and state variables"; Parameter10 "Bring state variables to output"; codeupdate "update code from mask"
      mask help: This is a level-2 MATLAB file S-function which demonstrates CISIA entity
      mask DialogControl Container1 Prompt: All parameters
      mask Display: image('Icons/Optical_Wire.png')
  Wire_2b (97) : M-S-Function  FunctionName=cisia_msfun  Parameters=Parameter1, Parameter2, Parameter3, resources, Parameter10, codeupdate, step_received, step_computed, dynamic_computed, step_sended, id_entity, id_project, id_type, name_type, color  mask(S-function:msfcn_unit_delay){Parameter1='Wire_2b', Parameter2=1, Parameter3='ORO', resources=, Parameter10=off, codeupdate=off, step_received=|, step_computed=, dynamic_computed=, step_sended=|, id_entity=97, id_project=6, id_type=1, name_type=Optical_Wire, color=#99CCFF}
      mask step_received=|
      | Connection=max(Connection_init,TLC_CONN);
      | TLC_services=max(TLC_services_init,TLC_SERVICE);
      | TLC_services=mod(TLC_services,10);
      | TLC_revoke=floor(TLC_SERVICE/10);
      |
      | Cyber_Fault=CYBER_FAULT;
      |
      | Mechanical_Fault=max([Mechanical_Fault MECH_FAULT Mechanical_Fault_init]);
      |
      | %TLC_services=TLC_services.*(1-TLC_revoke);
      |
      | Operative_Level=1-Mechanical_Fault;
      mask step_sended=|
      | TLC_CONN=Connection*Operative_Level;
      | TLC_SERVICE=TLC_services*Operative_Level+TLC_revoke*10;
      |
      |
      | CYBER_FAULT=Cyber_Fault*Operative_Level;
      | MECH_FAULT=Mechanical_Fault;
      mask prompts: Parameter1 "entity name"; Parameter2 "sampling time"; Parameter3 "project"; resources "input resources and state variables"; Parameter10 "Bring state variables to output"; codeupdate "update code from mask"
      mask help: This is a level-2 MATLAB file S-function which demonstrates CISIA entity
      mask DialogControl Container1 Prompt: All parameters
      mask Display: image('Icons/Optical_Wire.png')
  Wire_4 (12) : M-S-Function  FunctionName=cisia_msfun  Parameters=Parameter1, Parameter2, Parameter3, resources, Parameter10, codeupdate, step_received, step_computed, dynamic_computed, step_sended, id_entity, id_project, id_type, name_type, color  mask(S-function:msfcn_unit_delay){Parameter1='Wire_4', Parameter2=1, Parameter3='ORO', resources=, Parameter10=off, codeupdate=off, step_received=|, step_computed=, dynamic_computed=, step_sended=|, id_entity=12, id_project=6, id_type=1, name_type=Optical_Wire, color=#99CCFF}
      mask step_received=|
      | Connection=max(Connection_init,TLC_CONN);
      | TLC_services=max(TLC_services_init,TLC_SERVICE);
      | TLC_services=mod(TLC_services,10);
      | TLC_revoke=floor(TLC_SERVICE/10);
      |
      | Cyber_Fault=CYBER_FAULT;
      |
      | Mechanical_Fault=max([Mechanical_Fault MECH_FAULT Mechanical_Fault_init]);
      |
      | %TLC_services=TLC_services.*(1-TLC_revoke);
      |
      | Operative_Level=1-Mechanical_Fault;
      mask step_sended=|
      | TLC_CONN=Connection*Operative_Level;
      | TLC_SERVICE=TLC_services*Operative_Level+TLC_revoke*10;
      |
      |
      | CYBER_FAULT=Cyber_Fault*Operative_Level;
      | MECH_FAULT=Mechanical_Fault;
      mask prompts: Parameter1 "entity name"; Parameter2 "sampling time"; Parameter3 "project"; resources "input resources and state variables"; Parameter10 "Bring state variables to output"; codeupdate "update code from mask"
      mask help: This is a level-2 MATLAB file S-function which demonstrates CISIA entity
      mask DialogControl Container1 Prompt: All parameters
      mask Display: image('Icons/Optical_Wire.png')
  Wire_4b (13) : M-S-Function  FunctionName=cisia_msfun  Parameters=Parameter1, Parameter2, Parameter3, resources, Parameter10, codeupdate, step_received, step_computed, dynamic_computed, step_sended, id_entity, id_project, id_type, name_type, color  mask(S-function:msfcn_unit_delay){Parameter1='Wire_4b', Parameter2=1, Parameter3='ORO', resources=, Parameter10=off, codeupdate=off, step_received=|, step_computed=, dynamic_computed=, step_sended=|, id_entity=13, id_project=6, id_type=1, name_type=Optical_Wire, color=#99CCFF}
      mask step_received=|
      | Connection=max(Connection_init,TLC_CONN);
      | TLC_services=max(TLC_services_init,TLC_SERVICE);
      | TLC_services=mod(TLC_services,10);
      | TLC_revoke=floor(TLC_SERVICE/10);
      |
      | Cyber_Fault=CYBER_FAULT;
      |
      | Mechanical_Fault=max([Mechanical_Fault MECH_FAULT Mechanical_Fault_init]);
      |
      | %TLC_services=TLC_services.*(1-TLC_revoke);
      |
      | Operative_Level=1-Mechanical_Fault;
      mask step_sended=|
      | TLC_CONN=Connection*Operative_Level;
      | TLC_SERVICE=TLC_services*Operative_Level+TLC_revoke*10;
      |
      |
      | CYBER_FAULT=Cyber_Fault*Operative_Level;
      | MECH_FAULT=Mechanical_Fault;
      mask prompts: Parameter1 "entity name"; Parameter2 "sampling time"; Parameter3 "project"; resources "input resources and state variables"; Parameter10 "Bring state variables to output"; codeupdate "update code from mask"
      mask help: This is a level-2 MATLAB file S-function which demonstrates CISIA entity
      mask DialogControl Container1 Prompt: All parameters
      mask Display: image('Icons/Optical_Wire.png')
  Wire_6 (17) : M-S-Function  FunctionName=cisia_msfun  Parameters=Parameter1, Parameter2, Parameter3, resources, Parameter10, codeupdate, step_received, step_computed, dynamic_computed, step_sended, id_entity, id_project, id_type, name_type, color  mask(S-function:msfcn_unit_delay){Parameter1='Wire_6', Parameter2=1, Parameter3='ORO', resources=, Parameter10=off, codeupdate=off, step_received=|, step_computed=, dynamic_computed=, step_sended=|, id_entity=17, id_project=6, id_type=1, name_type=Optical_Wire, color=#99CCFF}
      mask step_received=|
      | Connection=max(Connection_init,TLC_CONN);
      | TLC_services=max(TLC_services_init,TLC_SERVICE);
      | TLC_services=mod(TLC_services,10);
      | TLC_revoke=floor(TLC_SERVICE/10);
      |
      | Cyber_Fault=CYBER_FAULT;
      |
      | Mechanical_Fault=max([Mechanical_Fault MECH_FAULT Mechanical_Fault_init]);
      |
      | %TLC_services=TLC_services.*(1-TLC_revoke);
      |
      | Operative_Level=1-Mechanical_Fault;
      mask step_sended=|
      | TLC_CONN=Connection*Operative_Level;
      | TLC_SERVICE=TLC_services*Operative_Level+TLC_revoke*10;
      |
      |
      | CYBER_FAULT=Cyber_Fault*Operative_Level;
      | MECH_FAULT=Mechanical_Fault;
      mask prompts: Parameter1 "entity name"; Parameter2 "sampling time"; Parameter3 "project"; resources "input resources and state variables"; Parameter10 "Bring state variables to output"; codeupdate "update code from mask"
      mask help: This is a level-2 MATLAB file S-function which demonstrates CISIA entity
      mask DialogControl Container1 Prompt: All parameters
      mask Display: image('Icons/Optical_Wire.png')
  Wire_6b (18) : M-S-Function  FunctionName=cisia_msfun  Parameters=Parameter1, Parameter2, Parameter3, resources, Parameter10, codeupdate, step_received, step_computed, dynamic_computed, step_sended, id_entity, id_project, id_type, name_type, color  mask(S-function:msfcn_unit_delay){Parameter1='Wire_6b', Parameter2=1, Parameter3='ORO', resources=, Parameter10=off, codeupdate=off, step_received=|, step_computed=, dynamic_computed=, step_sended=|, id_entity=18, id_project=6, id_type=1, name_type=Optical_Wire, color=#99CCFF}
      mask step_received=|
      | Connection=max(Connection_init,TLC_CONN);
      | TLC_services=max(TLC_services_init,TLC_SERVICE);
      | TLC_services=mod(TLC_services,10);
      | TLC_revoke=floor(TLC_SERVICE/10);
      |
      | Cyber_Fault=CYBER_FAULT;
      |
      | Mechanical_Fault=max([Mechanical_Fault MECH_FAULT Mechanical_Fault_init]);
      |
      | %TLC_services=TLC_services.*(1-TLC_revoke);
      |
      | Operative_Level=1-Mechanical_Fault;
      mask step_sended=|
      | TLC_CONN=Connection*Operative_Level;
      | TLC_SERVICE=TLC_services*Operative_Level+TLC_revoke*10;
      |
      |
      | CYBER_FAULT=Cyber_Fault*Operative_Level;
      | MECH_FAULT=Mechanical_Fault;
      mask prompts: Parameter1 "entity name"; Parameter2 "sampling time"; Parameter3 "project"; resources "input resources and state variables"; Parameter10 "Bring state variables to output"; codeupdate "update code from mask"
      mask help: This is a level-2 MATLAB file S-function which demonstrates CISIA entity
      mask DialogControl Container1 Prompt: All parameters
      mask Display: image('Icons/Optical_Wire.png')
  Wire_7 (19) : M-S-Function  FunctionName=cisia_msfun  Parameters=Parameter1, Parameter2, Parameter3, resources, Parameter10, codeupdate, step_received, step_computed, dynamic_computed, step_sended, id_entity, id_project, id_type, name_type, color  mask(S-function:msfcn_unit_delay){Parameter1='Wire_7', Parameter2=1, Parameter3='ORO', resources=, Parameter10=off, codeupdate=off, step_received=|, step_computed=, dynamic_computed=, step_sended=|, id_entity=19, id_project=6, id_type=1, name_type=Optical_Wire, color=#99CCFF}
      mask step_received=|
      | Connection=max(Connection_init,TLC_CONN);
      | TLC_services=max(TLC_services_init,TLC_SERVICE);
      | TLC_services=mod(TLC_services,10);
      | TLC_revoke=floor(TLC_SERVICE/10);
      |
      | Cyber_Fault=CYBER_FAULT;
      |
      | Mechanical_Fault=max([Mechanical_Fault MECH_FAULT Mechanical_Fault_init]);
      |
      | %TLC_services=TLC_services.*(1-TLC_revoke);
      |
      | Operative_Level=1-Mechanical_Fault;
      mask step_sended=|
      | TLC_CONN=Connection*Operative_Level;
      | TLC_SERVICE=TLC_services*Operative_Level+TLC_revoke*10;
      |
      |
      | CYBER_FAULT=Cyber_Fault*Operative_Level;
      | MECH_FAULT=Mechanical_Fault;
      mask prompts: Parameter1 "entity name"; Parameter2 "sampling time"; Parameter3 "project"; resources "input resources and state variables"; Parameter10 "Bring state variables to output"; codeupdate "update code from mask"
      mask help: This is a level-2 MATLAB file S-function which demonstrates CISIA entity
      mask DialogControl Container1 Prompt: All parameters
      mask Display: image('Icons/Optical_Wire.png')
  Wire_7b (20) : M-S-Function  FunctionName=cisia_msfun  Parameters=Parameter1, Parameter2, Parameter3, resources, Parameter10, codeupdate, step_received, step_computed, dynamic_computed, step_sended, id_entity, id_project, id_type, name_type, color  mask(S-function:msfcn_unit_delay){Parameter1='Wire_7b', Parameter2=1, Parameter3='ORO', resources=, Parameter10=off, codeupdate=off, step_received=|, step_computed=, dynamic_computed=, step_sended=|, id_entity=20, id_project=6, id_type=1, name_type=Optical_Wire, color=#99CCFF}
      mask step_received=|
      | Connection=max(Connection_init,TLC_CONN);
      | TLC_services=max(TLC_services_init,TLC_SERVICE);
      | TLC_services=mod(TLC_services,10);
      | TLC_revoke=floor(TLC_SERVICE/10);
      |
      | Cyber_Fault=CYBER_FAULT;
      |
      | Mechanical_Fault=max([Mechanical_Fault MECH_FAULT Mechanical_Fault_init]);
      |
      | %TLC_services=TLC_services.*(1-TLC_revoke);
      |
      | Operative_Level=1-Mechanical_Fault;
      mask step_sended=|
      | TLC_CONN=Connection*Operative_Level;
      | TLC_SERVICE=TLC_services*Operative_Level+TLC_revoke*10;
      |
      |
      | CYBER_FAULT=Cyber_Fault*Operative_Level;
      | MECH_FAULT=Mechanical_Fault;
      mask prompts: Parameter1 "entity name"; Parameter2 "sampling time"; Parameter3 "project"; resources "input resources and state variables"; Parameter10 "Bring state variables to output"; codeupdate "update code from mask"
      mask help: This is a level-2 MATLAB file S-function which demonstrates CISIA entity
      mask DialogControl Container1 Prompt: All parameters
      mask Display: image('Icons/Optical_Wire.png')
  Wire_8 (21) : M-S-Function  FunctionName=cisia_msfun  Parameters=Parameter1, Parameter2, Parameter3, resources, Parameter10, codeupdate, step_received, step_computed, dynamic_computed, step_sended, id_entity, id_project, id_type, name_type, color  mask(S-function:msfcn_unit_delay){Parameter1='Wire_8', Parameter2=1, Parameter3='ORO', resources=, Parameter10=off, codeupdate=off, step_received=|, step_computed=, dynamic_computed=, step_sended=|, id_entity=21, id_project=6, id_type=1, name_type=Optical_Wire, color=#99CCFF}
      mask step_received=|
      | Connection=max(Connection_init,TLC_CONN);
      | TLC_services=max(TLC_services_init,TLC_SERVICE);
      | TLC_services=mod(TLC_services,10);
      | TLC_revoke=floor(TLC_SERVICE/10);
      |
      | Cyber_Fault=CYBER_FAULT;
      |
      | Mechanical_Fault=max([Mechanical_Fault MECH_FAULT Mechanical_Fault_init]);
      |
      | %TLC_services=TLC_services.*(1-TLC_revoke);
      |
      | Operative_Level=1-Mechanical_Fault;
      mask step_sended=|
      | TLC_CONN=Connection*Operative_Level;
      | TLC_SERVICE=TLC_services*Operative_Level+TLC_revoke*10;
      |
      |
      | CYBER_FAULT=Cyber_Fault*Operative_Level;
      | MECH_FAULT=Mechanical_Fault;
      mask prompts: Parameter1 "entity name"; Parameter2 "sampling time"; Parameter3 "project"; resources "input resources and state variables"; Parameter10 "Bring state variables to output"; codeupdate "update code from mask"
      mask help: This is a level-2 MATLAB file S-function which demonstrates CISIA entity
      mask DialogControl Container1 Prompt: All parameters
      mask Display: image('Icons/Optical_Wire.png')
  Wire_8b (22) : M-S-Function  FunctionName=cisia_msfun  Parameters=Parameter1, Parameter2, Parameter3, resources, Parameter10, codeupdate, step_received, step_computed, dynamic_computed, step_sended, id_entity, id_project, id_type, name_type, color  mask(S-function:msfcn_unit_delay){Parameter1='Wire_8b', Parameter2=1, Parameter3='ORO', resources=, Parameter10=off, codeupdate=off, step_received=|, step_computed=, dynamic_computed=, step_sended=|, id_entity=22, id_project=6, id_type=1, name_type=Optical_Wire, color=#99CCFF}
      mask step_received=|
      | Connection=max(Connection_init,TLC_CONN);
      | TLC_services=max(TLC_services_init,TLC_SERVICE);
      | TLC_services=mod(TLC_services,10);
      | TLC_revoke=floor(TLC_SERVICE/10);
      |
      | Cyber_Fault=CYBER_FAULT;
      |
      | Mechanical_Fault=max([Mechanical_Fault MECH_FAULT Mechanical_Fault_init]);
      |
      | %TLC_services=TLC_services.*(1-TLC_revoke);
      |
      | Operative_Level=1-Mechanical_Fault;
      mask step_sended=|
      | TLC_CONN=Connection*Operative_Level;
      | TLC_SERVICE=TLC_services*Operative_Level+TLC_revoke*10;
      |
      |
      | CYBER_FAULT=Cyber_Fault*Operative_Level;
      | MECH_FAULT=Mechanical_Fault;
      mask prompts: Parameter1 "entity name"; Parameter2 "sampling time"; Parameter3 "project"; resources "input resources and state variables"; Parameter10 "Bring state variables to output"; codeupdate "update code from mask"
      mask help: This is a level-2 MATLAB file S-function which demonstrates CISIA entity
      mask DialogControl Container1 Prompt: All parameters
      mask Display: image('Icons/Optical_Wire.png')
  media3 : MATLAB Function  TreatAsAtomicUnit=on
  media4 : MATLAB Function  TreatAsAtomicUnit=on
  media5 : MATLAB Function  TreatAsAtomicUnit=on
  media6 : MATLAB Function  TreatAsAtomicUnit=on
  media7 : MATLAB Function  TreatAsAtomicUnit=on
  media8 : MATLAB Function  TreatAsAtomicUnit=on
  wires:
  Wire_8 (21)/4 -> Wire_8b (22)/4  "MECH_FAULT"
  media7/1(y) -> SAVE_5 (5)/1, Subsystem4/2(2)  "ROUTING_QoS"
  ASR920_1 (7)/4 -> [Routing_QoS_920_1]  "ROUTING_QoS"
  ASR9006_2 (10)/2 -> Wire_7 (19)/2, Wire_2b (97)/2  "TLC_SERVICE"
  [Routing_QoS_9006_1] -> Mux/1
  Wire_14 (42)/4 -> Wire_14b (43)/4  "MECH_FAULT"
  Subsystem/1(MEAN) -> SAVE_1 (3)/1, Display16/1  "IREWALL_GLOBAL_QoS"
  Wire_7b (20)/4 -> Wire_7 (19)/4  "MECH_FAULT"
  ASR920_1 (7)/2 -> 5G_CU_DU_Server_1 (160)/2, Wire_6b (18)/2  "TLC_SERVICE"
  Wire_8b (22)/4 -> Wire_8 (21)/4  "MECH_FAULT"
  Wire_12 (38)/4 -> Wire_12b (39)/4  "MECH_FAULT"
  ASR9006_1 (9)/4 -> [Routing_QoS_9006_1]  "ROUTING_QoS"
  Wire_4 (12)/4 -> Wire_4b (13)/4  "MECH_FAULT"
  [POWER_1] -> ASR9006_1 (9)/4  "POWER"
  Wire_7 (19)/4 -> Wire_7b (20)/4  "MECH_FAULT"
  FG1500_2 (33)/4 -> [FW_QoS_1]  "FIREWALL_QoS"
  [FW_QoS_2] -> Display17/1, Subsystem/2(2)
  Nex_1 (3)/2 -> ROUTE_ORO_1 (24)/1  "TLC_SERVICE"
  [Room_QoS_2] -> Nex_2 (4)/5  "ROOM_QoS"
  [Room_QoS_2] -> ASR9006_2 (10)/5  "ROOM_QoS"
  [Room_QoS_1] -> Nex_1 (3)/5  "ROOM_QoS"
  [Room_QoS_1] -> BIGP_2 (35)/5, FG1500_2 (33)/5  "ROOM_QoS"
  Nex_1 (3)/1 -> Wire_12 (38)/1, Wire_14 (42)/1, Wire_8 (21)/1, Wire_2 (2)/1, R_Wire_1 (98)/1  "TLC_CONN"
  Wire_12b (39)/4 -> Wire_12 (38)/4  "MECH_FAULT"
  BIGP_2 (35)/3 -> Wire_14b (43)/3  "CYBER_FAULT"
  Nex_2 (4)/2 -> ROUTE_ORO_2 (25)/1  "TLC_SERVICE"
  Subsystem3/1(MEAN) -> SAVE_6 (6)/1, Subsystem4/1(1)  "SWITCHING_QoS"
  Wire_6 (17)/4 -> Wire_6b (18)/4  "MECH_FAULT"
  [Redundancy_QoS_FG1500_1] -> Subsystem5/1(1)
  [POWER_2] -> ASR9006_2 (10)/4  "POWER"
  FG1500_2 (33)/5 -> [Redundancy_QoS_FG1500_2]  "REDUNDANCY_QoS"
  [Switching_QoS_Nex_2] -> Subsystem3/2(2)
  Subsystem5/1(MEAN) -> SAVE_7 (7)/1, Subsystem6/1(1)  "REDUNDANCY_QoS"
  Subsystem4/1(MEAN) -> SAVE_4 (4)/1, Subsystem6/2(2)  "MPLS_NET_QoS"
  BIGP_2 (35)/1 -> Wire_14b (43)/1  "TLC_CONN"
  TLC_service2/1 -> Nex_1 (3)/2  "TLC_SERVICE"
  TLC_service1/1 -> Nex_2 (4)/2  "TLC_SERVICE"
  TLC_conn2/1 -> Nex_1 (3)/1  "TLC_CONN"
  Wire_14b (43)/4 -> Wire_14 (42)/4  "MECH_FAULT"
  Alcatel_1 (26)/1 -> 5G_Core_1 (198)/1  "TLC_CONN"
  ASR9006_1 (9)/2 -> Wire_1b (96)/2, Wire_8b (22)/2, Wire_4b (13)/2  "TLC_SERVICE"
  ASR9006_2 (10)/1 -> Wire_7 (19)/1, Wire_2b (97)/1  "TLC_CONN"
  ASR9006_1 (9)/3 -> Wire_4b (13)/3, Wire_1b (96)/3, Wire_8b (22)/3  "CYBER_FAULT"
  ASR9006_1 (9)/1 -> Wire_4b (13)/1, Wire_1b (96)/1, Wire_8b (22)/1  "TLC_CONN"
  ASR920_1 (7)/1 -> 5G_CU_DU_Server_1 (160)/1, Wire_6b (18)/1  "TLC_CONN"
  CYBER_fault2/1 -> Nex_1 (3)/3  "CYBER_FAULT"
  media8/1(y) -> SAVE_2 (2)/1, Subsystem6/3(3)  "SERVICES_QoS"
  R_Wire_1 (98)/2 -> TLC_service1/1  "TLC_SERVICE"
  [Redundancy_QoS_FG1500_2] -> Subsystem5/2(2)
  [Room_QoS_1] -> ASR9006_1 (9)/5  "ROOM_QoS"
  ASR9006_2 (10)/4 -> [Routing_QoS_9006_2]  "ROUTING_QoS"
  [POWER_1] -> Nex_1 (3)/4  "POWER"
  [POWER_2] -> Nex_2 (4)/4  "POWER"
  [POWER_1] -> BIGP_2 (35)/4, FG1500_2 (33)/4  "POWER"
  TLC_conn1/1 -> Nex_2 (4)/1  "TLC_CONN"
  ASR903_1 (5)/4 -> [Routing_QoS_903_1]  "ROUTING_QoS"
  ASR920_1 (7)/3 -> 5G_CU_DU_Server_1 (160)/3, Wire_6b (18)/3  "CYBER_FAULT"
  FG1500_2 (33)/1 -> Wire_12b (39)/1  "TLC_CONN"
  Wire_6b (18)/4 -> Wire_6 (17)/4  "MECH_FAULT"
  FG1500_2 (33)/3 -> Wire_12b (39)/3  "CYBER_FAULT"
  [Switching_QoS_Nex_1] -> Subsystem3/1(1)
  [FW_QoS_1] -> Display9/1, Subsystem/1(1)
  Alcatel_1 (26)/2 -> 5G_Core_1 (198)/2  "TLC_SERVICE"
  Wire_4b (13)/4 -> Wire_4 (12)/4  "MECH_FAULT"
  R_Wire_1 (98)/1 -> TLC_conn1/1  "TLC_CONN"
  Alcatel_1 (26)/3 -> 5G_Core_1 (198)/3  "CYBER_FAULT"
  ROUTE_ORO_1 (24)/1 -> R_Wire_1 (98)/2  "TLC_SERVICE"
  Subsystem6/1(MEAN) -> SAVE_8 (8)/1  "GLOBAL_QoS"
  R_Wire_1b (99)/4 -> R_Wire_1 (98)/4  "MECH_FAULT"
  R_Wire_1 (98)/4 -> R_Wire_1b (99)/4  "MECH_FAULT"
  Nex_1 (3)/4 -> [Switching_QoS_Nex_1]  "SWITCHING_QoS"
  Nex_2 (4)/4 -> [Switching_QoS_Nex_2]  "SWITCHING_QoS"
  Wire_1b (96)/4 -> Wire_1 (1)/4  "MECH_FAULT"
  Wire_1 (1)/4 -> Wire_1b (96)/4  "MECH_FAULT"
  Wire_2b (97)/4 -> Wire_2 (2)/4  "MECH_FAULT"
  Wire_2 (2)/4 -> Wire_2b (97)/4  "MECH_FAULT"
  Wire_15a (49)/4 -> Wire_15 (44)/4  "MECH_FAULT"
  Wire_15 (44)/4 -> Wire_15a (49)/4  "MECH_FAULT"
  CYBER_fault1/1 -> Nex_2 (4)/3  "CYBER_FAULT"
  TLC_conn3/1 -> ASR9006_2 (10)/1  "TLC_CONN"
  TLC_service3/1 -> ASR9006_2 (10)/2  "TLC_SERVICE"
  CYBER_fault3/1 -> ASR9006_2 (10)/3  "CYBER_FAULT"
  TLC_conn4/1 -> ASR9006_1 (9)/1  "TLC_CONN"
  TLC_service4/1 -> ASR9006_1 (9)/2  "TLC_SERVICE"
  CYBER_fault4/1 -> ASR9006_1 (9)/3  "CYBER_FAULT"
  TLC_conn5/1 -> ASR903_1 (5)/1  "TLC_CONN"
  TLC_service5/1 -> ASR903_1 (5)/2  "TLC_SERVICE"
  CYBER_fault5/1 -> ASR903_1 (5)/3  "CYBER_FAULT"
  TLC_conn8/1 -> ASR920_1 (7)/1  "TLC_CONN"
  TLC_service8/1 -> ASR920_1 (7)/2  "TLC_SERVICE"
  CYBER_fault8/1 -> ASR920_1 (7)/3  "CYBER_FAULT"
  Room_6 (241)/1 -> 5G_Core_1 (198)/5, Building_3 (215)/1, Alcatel_1 (26)/5  "ROOM_QoS"
  PowerGen_3 (157)/1 -> Alcatel_1 (26)/4, Room_6 (241)/1, 5G_Core_1 (198)/4  "POWER"
  TLC_conn9/1 -> Alcatel_1 (26)/1  "TLC_CONN"
  5G_Core_1 (198)/1 -> TLC_conn9/1  "TLC_CONN"
  5G_Core_1 (198)/2 -> TLC_service9/1  "TLC_SERVICE"
  5G_Core_1 (198)/3 -> CYBER_fault9/1  "CYBER_FAULT"
  Wire_4b (13)/1 -> TLC_conn5/1  "TLC_CONN"
  Wire_4b (13)/3 -> CYBER_fault5/1  "CYBER_FAULT"
  Wire_8 (21)/1 -> TLC_conn4/1  "TLC_CONN"
  Wire_8 (21)/2 -> TLC_service4/1  "TLC_SERVICE"
  Wire_8 (21)/3 -> CYBER_fault4/1  "CYBER_FAULT"
  Wire_1 (1)/1 -> TLC_conn4/2  "TLC_CONN"
  Wire_1 (1)/2 -> TLC_service4/2  "TLC_SERVICE"
  Wire_1 (1)/3 -> CYBER_fault4/2  "CYBER_FAULT"
  Wire_4 (12)/1 -> TLC_conn4/3  "TLC_CONN"
  Wire_4 (12)/2 -> TLC_service4/3  "TLC_SERVICE"
  Wire_4 (12)/3 -> CYBER_fault4/3  "CYBER_FAULT"
  Wire_6 (17)/1 -> TLC_conn8/1  "TLC_CONN"
  Wire_6 (17)/2 -> TLC_service8/1  "TLC_SERVICE"
  Wire_6 (17)/3 -> CYBER_fault8/1  "CYBER_FAULT"
  Room_3 (200)/1 -> 5G_CU_DU_Server_1 (160)/5  "ROOM_QoS"
  PowerGen_4 (214)/1 -> [POWER_3], ASR920_1 (7)/4, Room_4 (237)/1, Room_3 (200)/1, 5G_CU_DU_Server_1 (160)/4  "POWER"
  5G_CU_DU_Server_1 (160)/1 -> TLC_conn8/4  "TLC_CONN"
  5G_CU_DU_Server_1 (160)/2 -> TLC_service8/4  "TLC_SERVICE"
  5G_CU_DU_Server_1 (160)/3 -> CYBER_fault8/4  "CYBER_FAULT"
  Room_1 (51)/1 -> Building_1 (53)/1, [Room_QoS_1]  "ROOM_QoS"
  PowerGen_1 (46)/1 -> [POWER_1], Room_1 (51)/1  "POWER"
  PowerGen_2 (47)/1 -> [POWER_2], Room_2 (52)/1  "POWER"
  Room_2 (52)/1 -> [Room_QoS_2], Building_2 (201)/1  "ROOM_QoS"
  R_Wire_1b (99)/1 -> TLC_conn2/1  "TLC_CONN"
  R_Wire_1b (99)/2 -> TLC_service2/1  "TLC_SERVICE"
  R_Wire_1b (99)/3 -> CYBER_fault2/1  "CYBER_FAULT"
  Nex_2 (4)/1 -> Wire_7b (20)/1, Wire_1 (1)/1, R_Wire_1b (99)/1  "TLC_CONN"
  ROUTE_ORO_2 (25)/1 -> R_Wire_1b (99)/2  "TLC_SERVICE"
  Nex_2 (4)/3 -> R_Wire_1b (99)/3, Wire_1 (1)/3, Wire_7b (20)/3  "CYBER_FAULT"
  Wire_7b (20)/1 -> TLC_conn3/1  "TLC_CONN"
  Wire_7b (20)/2 -> TLC_service3/1  "TLC_SERVICE"
  Wire_7b (20)/3 -> CYBER_fault3/1  "CYBER_FAULT"
  Wire_2 (2)/1 -> TLC_conn3/2  "TLC_CONN"
  Wire_2 (2)/2 -> TLC_service3/2  "TLC_SERVICE"
  Wire_2 (2)/3 -> CYBER_fault3/2  "CYBER_FAULT"
  ROUTE_ORO_1 (24)/2 -> Wire_8 (21)/2  "TLC_SERVICE"
  Nex_1 (3)/3 -> Wire_8 (21)/3, Wire_2 (2)/3, R_Wire_1 (98)/3, Wire_12 (38)/3, Wire_14 (42)/3  "CYBER_FAULT"
  ROUTE_ORO_1 (24)/3 -> Wire_2 (2)/2  "TLC_SERVICE"
  Wire_1b (96)/1 -> TLC_conn1/2  "TLC_CONN"
  ROUTE_ORO_2 (25)/2 -> Wire_1 (1)/2  "TLC_SERVICE"
  Wire_1b (96)/2 -> TLC_service1/2  "TLC_SERVICE"
  Wire_1b (96)/3 -> CYBER_fault1/2  "CYBER_FAULT"
  R_Wire_1 (98)/3 -> CYBER_fault1/1  "CYBER_FAULT"
  Wire_2b (97)/1 -> TLC_conn2/2  "TLC_CONN"
  Wire_2b (97)/2 -> TLC_service2/2  "TLC_SERVICE"
  Wire_2b (97)/3 -> CYBER_fault2/2  "CYBER_FAULT"
  Wire_8b (22)/1 -> TLC_conn2/3  "TLC_CONN"
  Wire_8b (22)/2 -> TLC_service2/3  "TLC_SERVICE"
  Wire_8b (22)/3 -> CYBER_fault2/3  "CYBER_FAULT"
  Wire_7 (19)/1 -> TLC_conn1/3  "TLC_CONN"
  Wire_7 (19)/2 -> TLC_service1/3  "TLC_SERVICE"
  Wire_7 (19)/3 -> CYBER_fault1/3  "CYBER_FAULT"
  ROUTE_ORO_2 (25)/3 -> Wire_7b (20)/2  "TLC_SERVICE"
  Room_4 (237)/1 -> ASR920_1 (7)/5  "ROOM_QoS"
  TLC_service9/1 -> Alcatel_1 (26)/2  "TLC_SERVICE"
  CYBER_fault9/1 -> Alcatel_1 (26)/3  "CYBER_FAULT"
  Room_7 (252)/1 -> ASR903_1 (5)/5  "ROOM_QoS"
  Alcatel_1 (26)/4 -> [Routing_QoS_Alcatel_1]  "ROUTING_QoS"
  Mux/1 -> media7/1(u)
  [Routing_QoS_9006_2] -> Mux/2
  [Routing_QoS_903_1] -> Mux/3
  [Routing_QoS_903_2] -> Mux/4
  [Routing_QoS_920_1] -> Mux/5
  [Routing_QoS_920_2] -> Mux/6
  [Routing_QoS_Alcatel_1] -> Mux/7
  [Routing_QoS_Alcatel_2] -> Mux/8
  Wire_4b (13)/2 -> TLC_service5/1  "TLC_SERVICE"
  [Mobile_QoS_1] -> Mux1/1
  [Mobile_QoS_2] -> Mux1/2
  [Building_QoS_1] -> Subsystem2/1(1)
  [Building_QoS_2] -> Subsystem2/2(2)
  Subsystem2/1(MEAN) -> SAVE_3 (3)/1  "BUILDING_QoS"
  Wire_12b (39)/1 -> TLC_conn2/4  "TLC_CONN"
  Wire_12b (39)/2 -> TLC_service2/4  "TLC_SERVICE"
  Wire_12b (39)/3 -> CYBER_fault2/4  "CYBER_FAULT"
  Wire_14b (43)/1 -> TLC_conn2/5  "TLC_CONN"
  Wire_14b (43)/2 -> TLC_service2/5  "TLC_SERVICE"
  Wire_14b (43)/3 -> CYBER_fault2/5  "CYBER_FAULT"
  TLC_conn12/1 -> BIGP_2 (35)/1  "TLC_CONN"
  TLC_service13/1 -> BIGP_2 (35)/2  "TLC_SERVICE"
  CYBER_fault13/1 -> BIGP_2 (35)/3  "CYBER_FAULT"
  TLC_conn11/1 -> FG1500_2 (33)/1  "TLC_CONN"
  TLC_service12/1 -> FG1500_2 (33)/2  "TLC_SERVICE"
  CYBER_fault12/1 -> FG1500_2 (33)/3  "CYBER_FAULT"
  Wire_12 (38)/1 -> TLC_conn11/1  "TLC_CONN"
  Wire_12 (38)/2 -> TLC_service12/1  "TLC_SERVICE"
  Wire_12 (38)/3 -> CYBER_fault12/1  "CYBER_FAULT"
  Wire_14 (42)/1 -> TLC_conn12/1  "TLC_CONN"
  Wire_14 (42)/2 -> TLC_service13/1  "TLC_SERVICE"
  Wire_14 (42)/3 -> CYBER_fault13/1  "CYBER_FAULT"
  ROUTE_ORO_1 (24)/4 -> Wire_12 (38)/2  "TLC_SERVICE"
  ROUTE_ORO_1 (24)/5 -> Wire_14 (42)/2  "TLC_SERVICE"
  [Routing_QoS_7606a] -> Mux/9
  FG1500_2 (33)/2 -> ROUTE_ORO_7 (38)/1  "TLC_SERVICE"
  BIGP_2 (35)/2 -> ROUTE_ORO_9 (40)/1  "TLC_SERVICE"
  ROUTE_ORO_9 (40)/1 -> Wire_14b (43)/2  "TLC_SERVICE"
  ROUTE_ORO_7 (38)/1 -> Wire_12b (39)/2  "TLC_SERVICE"
  Mux4/1 -> Display15/1, media4/1(u), Max/1
  Max/1 -> media5/1(u)
  media5/1(y) -> SAVE_22 (22)/1  "ALT_ALL"
  [Mobile_Alt_Serv_1] -> Mux3/2
  Mux5/1 -> media3/1(u), Max/3
  [Mobile_Alt_Rout_2] -> Mux4/3
  [Mobile_Alt_Rout_1] -> Mux4/2
  Mux3/1 -> Max/2, media6/1(u)
  [Mobile_Alt_Serv_2] -> Mux3/3
  media4/1(y) -> SAVE_20 (20)/1  "ALT_ROUTING"
  [Home_Alt_Serv_1] -> Mux3/1
  [Home_Alt_Rout_1] -> Mux4/1
  media6/1(y) -> SAVE_21 (21)/1  "ALT_SERVICES"
  [Home_Alt_Port_1] -> Mux5/1
  media3/1(y) -> SAVE_23 (23)/1  "ALT_PORT_ISOLATION"
  [Mobile_Alt_Port_1] -> Mux5/2
  [Mobile_Alt_Port_2] -> Mux5/3
  Splitter_1 (54)/1 -> ROUTE_ORO_4 (27)/1  "TLC_SERVICE"
  ONU_3 (282)/1 -> House_1 (145)/1  "TLC_SERVICE"
  ANTENNA_2 (60)/1 -> Mobile_2 (148)/1  "TLC_SERVICE"
  ANTENNA_1 (56)/3 -> Mobile_1 (147)/3  "R_CONN"
  ONU_1 (55)/3 -> ANTENNA_1 (56)/4  "NGPON_CONN"
  ONU_2 (58)/1 -> ANTENNA_2 (60)/1  "TLC_SERVICE"
  Mobile_1 (147)/4 -> [Mobile_Alt_Port_1]  "ALT_PORT_ISOLATION"
  Room_5 (240)/1 -> BLM_1500 (91)/5  "ROOM_QoS"
  Mobile_2 (148)/2 -> [Mobile_Alt_Rout_2]  "ALT_ROUTING"
  ONU_3 (282)/2 -> House_1 (145)/2  "CYBER_FAULT"
  House_1 (145)/1 -> [House_QoS_1]  "HOME_QoS"
  Mobile_2 (148)/3 -> [Mobile_Alt_Serv_2]  "ALT_SERVICES"
  Mobile_1 (147)/3 -> [Mobile_Alt_Serv_1]  "ALT_SERVICES"
  House_1 (145)/3 -> [Home_Alt_Serv_1]  "ALT_SERVICES"
  Mobile_1 (147)/2 -> [Mobile_Alt_Rout_1]  "ALT_ROUTING"
  BLM_1500 (91)/2 -> ROUTE_ORO_3 (26)/1  "TLC_SERVICE"
  BLM_1500 (91)/4 -> Splitter_1 (54)/3, [NGPON_CONN]  "NGPON_CONN"
  ONU_2 (58)/2 -> ANTENNA_2 (60)/2  "CYBER_FAULT"
  ANTENNA_2 (60)/3 -> Mobile_2 (148)/3  "R_CONN"
  ONU_2 (58)/3 -> ANTENNA_2 (60)/4  "NGPON_CONN"
  House_1 (145)/4 -> [Home_Alt_Port_1]  "ALT_PORT_ISOLATION"
  ROUTE_ORO_4 (27)/2 -> ONU_2 (58)/1  "TLC_SERVICE"
  ONU_1 (55)/2 -> ANTENNA_1 (56)/2  "CYBER_FAULT"
  BLM_1500 (91)/3 -> Splitter_1 (54)/2, Mask Port Saturation/1(IN)  "CYBER_FAULT"
  ROUTE_ORO_3 (26)/2 -> Splitter_1 (54)/1  "TLC_SERVICE"
  Splitter_1 (54)/3 -> ONU_3 (282)/4, ONU_2 (58)/4, ONU_1 (55)/4  "NGPON_CONN"
  Constant/1 -> ANTENNA_1 (56)/3, ANTENNA_2 (60)/3  "POWER"
  Splitter_1 (54)/2 -> ONU_3 (282)/2, ONU_2 (58)/2, ONU_1 (55)/2  "CYBER_FAULT"
  Splitter_1 (54)/4 -> BLM_1500 (91)/6  "NGPON_IN"
  Mobile_1 (147)/1 -> [Mobile_QoS_1]  "MOBILE_QoS"
  ROUTE_ORO_4 (27)/1 -> ONU_1 (55)/1  "TLC_SERVICE"
  ROUTE_ORO_4 (27)/3 -> ONU_3 (282)/1  "TLC_SERVICE"
  ANTENNA_1 (56)/1 -> Mobile_1 (147)/1  "TLC_SERVICE"
  ONU_3 (282)/3 -> House_1 (145)/4  "NGPON_CONN"
  ONU_1 (55)/1 -> ANTENNA_1 (56)/1  "TLC_SERVICE"
  ANTENNA_1 (56)/2 -> Mobile_1 (147)/2  "CYBER_FAULT"
  Mobile_2 (148)/4 -> [Mobile_Alt_Port_2]  "ALT_PORT_ISOLATION"
  Mobile_2 (148)/1 -> [Mobile_QoS_2]  "MOBILE_QoS"
  ANTENNA_2 (60)/2 -> Mobile_2 (148)/2  "CYBER_FAULT"
  House_1 (145)/2 -> [Home_Alt_Rout_1]  "ALT_ROUTING"
  PowerGen_5 (236)/1 -> ONU_1 (55)/3  "POWER"
  PowerGen_6 (245)/1 -> ONU_2 (58)/3  "POWER"
  PowerGen_7 (260)/1 -> House_1 (145)/3, ONU_3 (282)/3  "POWER"
  [POWER_3] -> BLM_1500 (91)/4, Room_5 (240)/1  "POWER"
  Wire_15 (44)/1 -> BLM_1500 (91)/1  "TLC_CONN"
  Wire_15 (44)/2 -> BLM_1500 (91)/2  "TLC_SERVICE"
  Wire_15 (44)/3 -> BLM_1500 (91)/3  "CYBER_FAULT"
  BLM_1500 (91)/1 -> Wire_15a (49)/1  "TLC_CONN"
  ROUTE_ORO_3 (26)/1 -> Wire_15a (49)/2  "TLC_SERVICE"
  Mask Port Saturation/1(OUT) -> Wire_15a (49)/3  "CYBER_FAULT"
  Mux1/1 -> media8/1(u)
  [House_QoS_1] -> Mux1/3
  Building_1 (53)/2 -> [Building_QoS_1]  "BUILDING_QoS"
  Building_2 (201)/2 -> [Building_QoS_2]  "BUILDING_QoS"
  Mask Port Saturation2/1(OUT) -> Wire_7 (19)/3, Wire_2b (97)/3  "CYBER_FAULT"
  Wire_10 (30)/4 -> Wire_10b (31)/4  "MECH_FAULT"
  Wire_10b (31)/4 -> Wire_10 (30)/4  "MECH_FAULT"
  CISIA_MASTER (0)/2 -> Display2/1  "MAJOR HITS"
  CISIA_MASTER (0)/1 -> Display1/1  "MINOR HITS"
  CISIA_MASTER (0)/3 -> Display3/1  "DELTA TIME"
  CISIA_MASTER (0)/4 -> Display4/1  "TIME PAST"
